simulink model "phantomx_sim_attitude"  (R2025b)
settings: Solver=daessc  StartTime=0.0  StopTime=20  RelTol=1e-3
InitFcn:
  | % Parametri del filtro
  | num_filters = 18;       % Numero di filtri in parallelo (i tuoi 18 giunti/segnali)
  | if evalin('base','exist(''tau_filtro'',''var'')')
  |     tau = evalin('base','tau_filtro');
  | else
  |     tau = 0.05; % costante di tempo del polo
  | end
  | a = 1 / tau;            % Polo del sistema
  | 
  | % 1. Creazione delle Matrici di Stato (State-Space)
  | % Matrice A (Dinamica del sistema): Diagonale con i poli
  | A = -a * eye(num_filters);
  | 
  | % Matrice B (Matrice di ingresso): Diagonale per mappare ogni input al suo stato
  | B = a * eye(num_filters);
  | 
  | % Matrice C (Matrice di uscita): Identità (vogliamo leggere gli stati direttamente)
  | C = eye(num_filters);
  | 
  | % Matrice D (Feedforward): Matrice di zeri (nessun collegamento diretto input-output)
  | D = zeros(num_filters, num_filters);
  | 
  | % 2. Creazione dell'oggetto State-Space in MATLAB
  | sys_filter = ss(A, B, C, D);
  | 
  | % Aggiungiamo i nomi per tenere tutto in ordine (opzionale ma consigliato)
  | sys_filter.InputName = strcat('Action_In_', string(1:num_filters));
  | sys_filter.OutputName = strcat('Filtered_Action_Out_', string(1:num_filters));
  | sys_filter.StateName = strcat('State_', string(1:num_filters));
  | 
  | % Mostra le proprietà del sistema creato
  | disp('Sistema State-Space creato con successo:');
  | sys_filter
  | 
  | run init_gait.m
values from neighbouring files (symbols this model uses):
  c2_par = [double(cfg.c2.attiva),            cfg.c2.z_nom,            cfg.c2.v_search,            cfg.c2.z_ext_max,            cfg.c2.t_reset,            cfg.c2.tol]    [init_gait.m]
  c2_soglia = inf    [init_gait.m]
undefined symbols (not defined in the file or in its folder): gait, X, Y, Z
libraries: sm_lib x305, nesl_utility x100, robotmaniplib x1, slpidlib x1
(part 1 of 5)
settings Model: Creator=andri  LastModifiedBy=eros2
settings SimscapeCC: SimscapeLogType=all  SimscapeLogLimitData=off

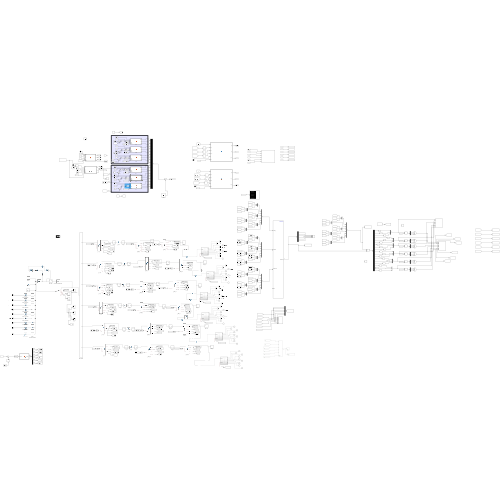
[thumbnail: Simulink's stored preview of the top-level diagram]
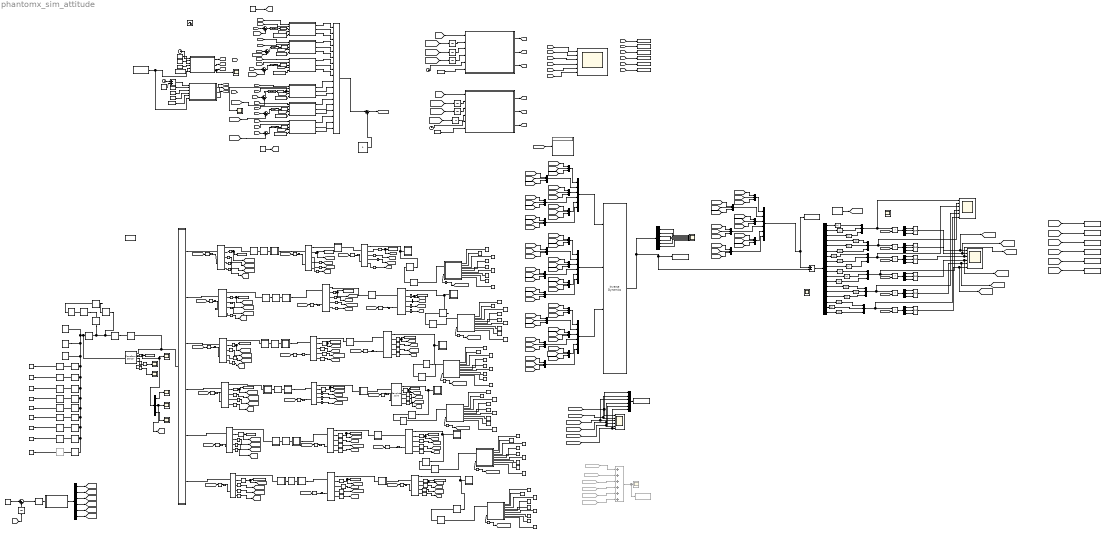
== system phantomx_sim_attitude ==
  note: LEFT
  note: RIGHT
  6-DOF Joint : sm_lib/Joints/6-DOF Joint  JointMode=Normal  CompositeWrenchDir=FollowerOnBase  CompositeWrenchFrame=BaseFrame  SenseConstraintForce=off  SenseConstraintTorque=off  SenseTotalForce=off  SenseTotalTorque=off  PxPositionTargetSpecify=off  PxPositionTargetPriority=High  PxPositionTargetValue=0  PxPositionTargetValueUnits=m  PxVelocityTargetSpecify=off  PxVelocityTargetPriority=High  PxVelocityTargetValue=0  PxVelocityTargetValueUnits=m/s  PxEquilibriumPosition=0  PxEquilibriumPositionUnits=m  PxSpringStiffness=0  PxSpringStiffnessUnits=N/m  PxDampingCoefficient=0  PxDampingCoefficientUnits=N/(m/s)  PxLowerLimitSpecify=off  PxLowerLimitBound=-1  PxLowerLimitBoundUnits=m  PxLowerLimitStiffness=1e6  PxLowerLimitStiffnessUnits=N/m  PxLowerLimitDamping=1e3  PxLowerLimitDampingUnits=N/(m/s)  PxLowerLimitTransitionRegionWidth=1e-4  PxLowerLimitTransitionRegionWidthUnits=m  PxUpperLimitSpecify=off  PxUpperLimitBound=1  PxUpperLimitBoundUnits=m  PxUpperLimitStiffness=1e6  PxUpperLimitStiffnessUnits=N/m  PxUpperLimitDamping=1e3  PxUpperLimitDampingUnits=N/(m/s)  PxUpperLimitTransitionRegionWidth=1e-4  PxUpperLimitTransitionRegionWidthUnits=m  PxTorqueActuationMode=NoTorque  PxMotionActuationMode=ComputedMotion  PxSensePosition=off  PxSenseVelocity=off  PxSenseAcceleration=off  PxSenseTorqueForce=off  PxSenseLowerLimitTorqueForce=off  PxSenseUpperLimitTorqueForce=off  PyPositionTargetSpecify=off  PyPositionTargetPriority=High  PyPositionTargetValue=0  PyPositionTargetValueUnits=m  PyVelocityTargetSpecify=off  PyVelocityTargetPriority=High  PyVelocityTargetValue=0  PyVelocityTargetValueUnits=m/s  PyEquilibriumPosition=0  PyEquilibriumPositionUnits=m  PySpringStiffness=0  PySpringStiffnessUnits=N/m  PyDampingCoefficient=0  PyDampingCoefficientUnits=N/(m/s)  PyLowerLimitSpecify=off  PyLowerLimitBound=-1  PyLowerLimitBoundUnits=m  PyLowerLimitStiffness=1e6  PyLowerLimitStiffnessUnits=N/m  PyLowerLimitDamping=1e3  PyLowerLimitDampingUnits=N/(m/s)  PyLowerLimitTransitionRegionWidth=1e-4  PyLowerLimitTransitionRegionWidthUnits=m  PyUpperLimitSpecify=off  PyUpperLimitBound=1  PyUpperLimitBoundUnits=m  PyUpperLimitStiffness=1e6  PyUpperLimitStiffnessUnits=N/m  PyUpperLimitDamping=1e3  PyUpperLimitDampingUnits=N/(m/s)  PyUpperLimitTransitionRegionWidth=1e-4  PyUpperLimitTransitionRegionWidthUnits=m  PyTorqueActuationMode=NoTorque  PyMotionActuationMode=ComputedMotion  PySensePosition=off  PySenseVelocity=off  PySenseAcceleration=off  PySenseTorqueForce=off  PySenseLowerLimitTorqueForce=off  PySenseUpperLimitTorqueForce=off  PzPositionTargetSpecify=on  PzPositionTargetPriority=High  PzPositionTargetValue=body_z0  PzPositionTargetValueUnits=m  PzVelocityTargetSpecify=off  PzVelocityTargetPriority=High  PzVelocityTargetValue=0  PzVelocityTargetValueUnits=m/s  PzEquilibriumPosition=0  PzEquilibriumPositionUnits=m  PzSpringStiffness=0  PzSpringStiffnessUnits=N/m  PzDampingCoefficient=0  PzDampingCoefficientUnits=N/(m/s)  PzLowerLimitSpecify=off  PzLowerLimitBound=-1  PzLowerLimitBoundUnits=m  PzLowerLimitStiffness=1e6  PzLowerLimitStiffnessUnits=N/m  PzLowerLimitDamping=1e3  PzLowerLimitDampingUnits=N/(m/s)  PzLowerLimitTransitionRegionWidth=1e-4  PzLowerLimitTransitionRegionWidthUnits=m  PzUpperLimitSpecify=off  PzUpperLimitBound=1  PzUpperLimitBoundUnits=m  PzUpperLimitStiffness=1e6  PzUpperLimitStiffnessUnits=N/m  PzUpperLimitDamping=1e3  PzUpperLimitDampingUnits=N/(m/s)  PzUpperLimitTransitionRegionWidth=1e-4  PzUpperLimitTransitionRegionWidthUnits=m  PzTorqueActuationMode=NoTorque  PzMotionActuationMode=ComputedMotion  PzSensePosition=off  PzSenseVelocity=off  PzSenseAcceleration=off  PzSenseTorqueForce=off  PzSenseLowerLimitTorqueForce=off  PzSenseUpperLimitTorqueForce=off  SphPositionTargetSpecify=off  SphPositionTargetPriority=High  SphPositionTargetRotationMethod=None  SphPositionTargetFollAlignAxisA=+X  SphPositionTargetBaseAlignAxisA=+Y  SphPositionTargetFollAlignAxisB=+Y  SphPositionTargetBaseAlignAxisB=+Z  SphPositionTargetRotationStandardAxis=+Z  SphPositionTargetRotationAngle=0  SphPositionTargetRotationAngleUnits=deg  SphPositionTargetRotationArbitraryAxis=[0 0 1]  SphPositionTargetRotationSequenceAxes=FollowerAxes  SphPositionTargetRotationSequence=XYX  SphPositionTargetRotationSequenceAngles=[0 0 0]  SphPositionTargetRotationSequenceAnglesUnits=deg  SphPositionTargetRotationMatrix=[1 0 0;0 1 0;0 0 1]  SphPositionTargetQuaternion=[1 0 0 0]  SphVelocityTargetSpecify=off  SphVelocityTargetPriority=High  SphVelocityTargetValue=[0 0 0]  SphVelocityTargetValueUnits=deg/s  SphVelocityTargetInFollowerFrame=on  SphEqPosRotationMethod=None  SphEqPosFollAlignAxisA=+X  SphEqPosBaseAlignAxisA=+Y  SphEqPosFollAlignAxisB=+Y  SphEqPosBaseAlignAxisB=+Z  SphEqPosRotationStandardAxis=+Z  SphEqPosRotationAngle=0  SphEqPosRotationAngleUnits=deg  SphEqPosRotationArbitraryAxis=[0 0 1]  SphEqPosRotationSequenceAxes=FollowerAxes  SphEqPosRotationSequence=XYX  SphEqPosRotationSequenceAngles=[0 0 0]  SphEqPosRotationSequenceAnglesUnits=deg  SphEqPosRotationMatrix=[1 0 0;0 1 0;0 0 1]  SphEqPosQuaternion=[1 0 0 0]  SphSpringStiffness=0  SphSpringStiffnessUnits=N*m/deg  SphDampingCoefficient=0  SphDampingCoefficientUnits=N*m/(deg/s)  SphLowerLimitSpecify=off  SphLowerLimitBound=15  SphLowerLimitBoundUnits=deg  SphLowerLimitStiffness=1e4  SphLowerLimitStiffnessUnits=N*m/deg  SphLowerLimitDamping=10  SphLowerLimitDampingUnits=N*m/(deg/s)  SphLowerLimitTransitionRegionWidth=0.1  SphLowerLimitTransitionRegionWidthUnits=deg  SphUpperLimitSpecify=off  SphUpperLimitBound=45  SphUpperLimitBoundUnits=deg  SphUpperLimitStiffness=1e4  SphUpperLimitStiffnessUnits=N*m/deg  SphUpperLimitDamping=10  SphUpperLimitDampingUnits=N*m/(deg/s)  SphUpperLimitTransitionRegionWidth=0.1  SphUpperLimitTransitionRegionWidthUnits=deg  SphTorqueActuationMode=NoTorque  SphActuateTorqueX=off  SphActuateTorqueY=off  SphActuateTorqueZ=off  SphActuateTorque=off  SphActuationFrame=BaseFrame  SphSensePosition=off  SphSenseVelocityX=off  SphSenseVelocityY=off  SphSenseVelocityZ=off  SphSenseVelocity=off  SphSenseAccelerationX=off  SphSenseAccelerationY=off  SphSenseAccelerationZ=off  SphSenseAcceleration=off  SphSenseLowerLimitTorqueMag=off  SphSenseUpperLimitTorqueMag=off  SphSensingFrame=BaseFrame
  6-DOF Joint1 : sm_lib/Joints/6-DOF Joint  JointMode=Normal  CompositeWrenchDir=FollowerOnBase  CompositeWrenchFrame=BaseFrame  SenseConstraintForce=off  SenseConstraintTorque=off  SenseTotalForce=off  SenseTotalTorque=off  PxPositionTargetSpecify=off  PxPositionTargetPriority=High  PxPositionTargetValue=0  PxPositionTargetValueUnits=m  PxVelocityTargetSpecify=off  PxVelocityTargetPriority=High  PxVelocityTargetValue=0  PxVelocityTargetValueUnits=m/s  PxEquilibriumPosition=0  PxEquilibriumPositionUnits=m  PxSpringStiffness=0  PxSpringStiffnessUnits=N/m  PxDampingCoefficient=0  PxDampingCoefficientUnits=N/(m/s)  PxLowerLimitSpecify=off  PxLowerLimitBound=-1  PxLowerLimitBoundUnits=m  PxLowerLimitStiffness=1e6  PxLowerLimitStiffnessUnits=N/m  PxLowerLimitDamping=1e3  PxLowerLimitDampingUnits=N/(m/s)  PxLowerLimitTransitionRegionWidth=1e-4  PxLowerLimitTransitionRegionWidthUnits=m  PxUpperLimitSpecify=off  PxUpperLimitBound=1  PxUpperLimitBoundUnits=m  PxUpperLimitStiffness=1e6  PxUpperLimitStiffnessUnits=N/m  PxUpperLimitDamping=1e3  PxUpperLimitDampingUnits=N/(m/s)  PxUpperLimitTransitionRegionWidth=1e-4  PxUpperLimitTransitionRegionWidthUnits=m  PxTorqueActuationMode=NoTorque  PxMotionActuationMode=ComputedMotion  PxSensePosition=off  PxSenseVelocity=off  PxSenseAcceleration=off  PxSenseTorqueForce=off  PxSenseLowerLimitTorqueForce=off  PxSenseUpperLimitTorqueForce=off  PyPositionTargetSpecify=off  PyPositionTargetPriority=High  PyPositionTargetValue=0  PyPositionTargetValueUnits=m  PyVelocityTargetSpecify=off  PyVelocityTargetPriority=High  PyVelocityTargetValue=0  PyVelocityTargetValueUnits=m/s  PyEquilibriumPosition=0  PyEquilibriumPositionUnits=m  PySpringStiffness=0  PySpringStiffnessUnits=N/m  PyDampingCoefficient=0  PyDampingCoefficientUnits=N/(m/s)  PyLowerLimitSpecify=off  PyLowerLimitBound=-1  PyLowerLimitBoundUnits=m  PyLowerLimitStiffness=1e6  PyLowerLimitStiffnessUnits=N/m  PyLowerLimitDamping=1e3  PyLowerLimitDampingUnits=N/(m/s)  PyLowerLimitTransitionRegionWidth=1e-4  PyLowerLimitTransitionRegionWidthUnits=m  PyUpperLimitSpecify=off  PyUpperLimitBound=1  PyUpperLimitBoundUnits=m  PyUpperLimitStiffness=1e6  PyUpperLimitStiffnessUnits=N/m  PyUpperLimitDamping=1e3  PyUpperLimitDampingUnits=N/(m/s)  PyUpperLimitTransitionRegionWidth=1e-4  PyUpperLimitTransitionRegionWidthUnits=m  PyTorqueActuationMode=NoTorque  PyMotionActuationMode=ComputedMotion  PySensePosition=off  PySenseVelocity=off  PySenseAcceleration=off  PySenseTorqueForce=off  PySenseLowerLimitTorqueForce=off  PySenseUpperLimitTorqueForce=off  PzPositionTargetSpecify=on  PzPositionTargetPriority=High  PzPositionTargetValue=body_z0  PzPositionTargetValueUnits=m  PzVelocityTargetSpecify=off  PzVelocityTargetPriority=High  PzVelocityTargetValue=0  PzVelocityTargetValueUnits=m/s  PzEquilibriumPosition=0  PzEquilibriumPositionUnits=m  PzSpringStiffness=0  PzSpringStiffnessUnits=N/m  PzDampingCoefficient=0  PzDampingCoefficientUnits=N/(m/s)  PzLowerLimitSpecify=off  PzLowerLimitBound=-1  PzLowerLimitBoundUnits=m  PzLowerLimitStiffness=1e6  PzLowerLimitStiffnessUnits=N/m  PzLowerLimitDamping=1e3  PzLowerLimitDampingUnits=N/(m/s)  PzLowerLimitTransitionRegionWidth=1e-4  PzLowerLimitTransitionRegionWidthUnits=m  PzUpperLimitSpecify=off  PzUpperLimitBound=1  PzUpperLimitBoundUnits=m  PzUpperLimitStiffness=1e6  PzUpperLimitStiffnessUnits=N/m  PzUpperLimitDamping=1e3  PzUpperLimitDampingUnits=N/(m/s)  PzUpperLimitTransitionRegionWidth=1e-4  PzUpperLimitTransitionRegionWidthUnits=m  PzTorqueActuationMode=NoTorque  PzMotionActuationMode=ComputedMotion  PzSensePosition=off  PzSenseVelocity=off  PzSenseAcceleration=off  PzSenseTorqueForce=off  PzSenseLowerLimitTorqueForce=off  PzSenseUpperLimitTorqueForce=off  SphPositionTargetSpecify=off  SphPositionTargetPriority=High  SphPositionTargetRotationMethod=None  SphPositionTargetFollAlignAxisA=+X  SphPositionTargetBaseAlignAxisA=+Y  SphPositionTargetFollAlignAxisB=+Y  SphPositionTargetBaseAlignAxisB=+Z  SphPositionTargetRotationStandardAxis=+Z  SphPositionTargetRotationAngle=0  SphPositionTargetRotationAngleUnits=deg  SphPositionTargetRotationArbitraryAxis=[0 0 1]  SphPositionTargetRotationSequenceAxes=FollowerAxes  SphPositionTargetRotationSequence=XYX  SphPositionTargetRotationSequenceAngles=[0 0 0]  SphPositionTargetRotationSequenceAnglesUnits=deg  SphPositionTargetRotationMatrix=[1 0 0;0 1 0;0 0 1]  SphPositionTargetQuaternion=[1 0 0 0]  SphVelocityTargetSpecify=off  SphVelocityTargetPriority=High  SphVelocityTargetValue=[0 0 0]  SphVelocityTargetValueUnits=deg/s  SphVelocityTargetInFollowerFrame=on  SphEqPosRotationMethod=None  SphEqPosFollAlignAxisA=+X  SphEqPosBaseAlignAxisA=+Y  SphEqPosFollAlignAxisB=+Y  SphEqPosBaseAlignAxisB=+Z  SphEqPosRotationStandardAxis=+Z  SphEqPosRotationAngle=0  SphEqPosRotationAngleUnits=deg  SphEqPosRotationArbitraryAxis=[0 0 1]  SphEqPosRotationSequenceAxes=FollowerAxes  SphEqPosRotationSequence=XYX  SphEqPosRotationSequenceAngles=[0 0 0]  SphEqPosRotationSequenceAnglesUnits=deg  SphEqPosRotationMatrix=[1 0 0;0 1 0;0 0 1]  SphEqPosQuaternion=[1 0 0 0]  SphSpringStiffness=0  SphSpringStiffnessUnits=N*m/deg  SphDampingCoefficient=0  SphDampingCoefficientUnits=N*m/(deg/s)  SphLowerLimitSpecify=off  SphLowerLimitBound=15  SphLowerLimitBoundUnits=deg  SphLowerLimitStiffness=1e4  SphLowerLimitStiffnessUnits=N*m/deg  SphLowerLimitDamping=10  SphLowerLimitDampingUnits=N*m/(deg/s)  SphLowerLimitTransitionRegionWidth=0.1  SphLowerLimitTransitionRegionWidthUnits=deg  SphUpperLimitSpecify=off  SphUpperLimitBound=45  SphUpperLimitBoundUnits=deg  SphUpperLimitStiffness=1e4  SphUpperLimitStiffnessUnits=N*m/deg  SphUpperLimitDamping=10  SphUpperLimitDampingUnits=N*m/(deg/s)  SphUpperLimitTransitionRegionWidth=0.1  SphUpperLimitTransitionRegionWidthUnits=deg  SphTorqueActuationMode=NoTorque  SphActuateTorqueX=off  SphActuateTorqueY=off  SphActuateTorqueZ=off  SphActuateTorque=off  SphActuationFrame=BaseFrame  SphSensePosition=off  SphSenseVelocityX=off  SphSenseVelocityY=off  SphSenseVelocityZ=off  SphSenseVelocity=off  SphSenseAccelerationX=off  SphSenseAccelerationY=off  SphSenseAccelerationZ=off  SphSenseAcceleration=off  SphSenseLowerLimitTorqueMag=off  SphSenseUpperLimitTorqueMag=off  SphSensingFrame=BaseFrame
  Abs{,1..17} (18 alike) : Abs  SaturateOnIntegerOverflow=off
  Add : Sum
  Add1 : Sum  Commented=on  Inputs=++++++
  Brick Solid : sm_lib/Body Elements/Brick Solid  BrickDimensions=[0.2 0.2 0.2]  BrickDimensionsUnits=m  ExportEntireGeometry=on  InertiaType=CalculateFromGeometry  BasedOnType=Mass  Density=1000  DensityUnits=kg/m^3  Mass=1  MassUnits=kg  CenterOfMass=[0 0 0]  CenterOfMassUnits=m  MomentsOfInertia=[1 1 1]  MomentsOfInertiaUnits=kg*m^2  ProductsOfInertia=[0 0 0]  ProductsOfInertiaUnits=kg*m^2  GraphicType=FromGeometry  MarkerShape=Sphere  MarkerSize=10  GraphicVisPropType=SimpleVisualProperties  GraphicDiffuseColor=[0.5 0.5 0.5]  GraphicOpacity=1  GraphicSpecularColor=[0.5 0.5 0.5 1.0]  GraphicAmbientColor=[0.15 0.15 0.15 1.0]  GraphicEmissiveColor=[0.0 0.0 0.0 1.0]  GraphicShininess=75  DoExposeReferenceFrame=on  SerializedFrames=<Frames/>
  Brick Solid1 : sm_lib/Body Elements/Brick Solid  BrickDimensions=[0.3 0.3 0.1]  BrickDimensionsUnits=m  ExportEntireGeometry=on  InertiaType=CalculateFromGeometry  BasedOnType=Mass  Density=1000  DensityUnits=kg/m^3  Mass=0.1  MassUnits=kg  CenterOfMass=[0 0 0]  CenterOfMassUnits=m  MomentsOfInertia=[1 1 1]  MomentsOfInertiaUnits=kg*m^2  ProductsOfInertia=[0 0 0]  ProductsOfInertiaUnits=kg*m^2  GraphicType=FromGeometry  MarkerShape=Sphere  MarkerSize=10  GraphicVisPropType=SimpleVisualProperties  GraphicDiffuseColor=[0.5 0.5 0.5]  GraphicOpacity=1  GraphicSpecularColor=[0.5 0.5 0.5 1.0]  GraphicAmbientColor=[0.15 0.15 0.15 1.0]  GraphicEmissiveColor=[0.0 0.0 0.0 1.0]  GraphicShininess=75  DoExposeReferenceFrame=on  SerializedFrames=<Frames/>
  Clock{,1..3} (4 alike) : Clock
  Connection Label{,1,4..5,27,45,54} (7 alike) : ConnectionLabel  Label=pavimento
  Connection Label{10,23..25,34,49,58} (7 alike) : ConnectionLabel  Label=ostacolo3
  Connection Label{3,7,11,26,35,50,59} (7 alike) : ConnectionLabel  Label=rampa
  Connection Label{6,12..14,28,46,55} (7 alike) : ConnectionLabel  Label=ostacolo7
  Connection Label{8,15,17..18,29,47,56} (7 alike) : ConnectionLabel  Label=ostacolo2
  Connection Label{2,9,16,19,30,48,57} (7 alike) : ConnectionLabel  Label=ostacolo1
  Connection Label{20,31..33,36,51,60} (7 alike) : ConnectionLabel  Label=ostacolo4
  Connection Label{21,37..38,40,42,52,61} (7 alike) : ConnectionLabel  Label=ostacolo5
  Connection Label{22,39,41,43..44,53,62} (7 alike) : ConnectionLabel  Label=ostacolo6
  Constant : Constant  Value=c2_soglia
  Constant1 : Constant  Value=gait.duty
  Constant10 : Constant  Value=c2_par
  Constant11 : Constant  Value=c2_par
  Constant12 : Constant  Value=0
  Constant19 : Constant  Value=deg2rad(-135)
  Constant2 : Constant  Value=gait.T
  Constant20 : Constant  Value=deg2rad(-90)
  Constant21 : Constant  Value=deg2rad(-45)
  Constant22 : Constant  Value=-1
  Constant23 : Constant
  Constant25 : Constant  Value=deg2rad(135)
  Constant26 : Constant  Value=deg2rad(90)
  Constant27 : Constant  Value=deg2rad(45)
  Constant28 : Constant  Value=0.5
  Constant3 : Constant  Value=gait.S
  Constant4 : Constant  Value=gait.H
  Constant5 : Constant  Value=gait.z0
  Constant6 : Constant  Value=gait.T
  Constant7 : Constant  Value=gait.S
  Constant8 : Constant  Value=gait.H
  Constant9 : Constant  Value=gait.z0
  Data Store Memory : DataStoreMemory  Priority=1  DataStoreName=joint_vector  WriteAfterWriteMsg=warning  InitialValue=zeros(21,1)  ShowAdditionalParam=off  OutDataTypeStr=double
  Data Store Write : DataStoreWrite  Priority=2  DataStoreName=joint_vector  DataStoreElements=joint_vector  EnableIndexing=on  IndexOptions=Index vector (dialog)  Indices=1  OutputSizes=1
  Data Store Write1 : DataStoreWrite  Priority=2  DataStoreName=joint_vector  DataStoreElements=joint_vector  EnableIndexing=on  IndexOptions=Index vector (dialog)  Indices=2  OutputSizes=1
  Data Store Write10 : DataStoreWrite  Priority=2  DataStoreName=joint_vector  DataStoreElements=joint_vector  EnableIndexing=on  IndexOptions=Index vector (dialog)  Indices=11  OutputSizes=1
  Data Store Write11 : DataStoreWrite  Priority=2  DataStoreName=joint_vector  DataStoreElements=joint_vector  EnableIndexing=on  IndexOptions=Index vector (dialog)  Indices=12  OutputSizes=1
  Data Store Write12 : DataStoreWrite  Priority=2  DataStoreName=joint_vector  DataStoreElements=joint_vector  EnableIndexing=on  IndexOptions=Index vector (dialog)  Indices=13  OutputSizes=1
  Data Store Write13 : DataStoreWrite  Priority=2  DataStoreName=joint_vector  DataStoreElements=joint_vector  EnableIndexing=on  IndexOptions=Index vector (dialog)  Indices=14  OutputSizes=1
  Data Store Write14 : DataStoreWrite  Priority=2  DataStoreName=joint_vector  DataStoreElements=joint_vector  EnableIndexing=on  IndexOptions=Index vector (dialog)  Indices=15  OutputSizes=1
  Data Store Write15 : DataStoreWrite  Priority=2  DataStoreName=joint_vector  DataStoreElements=joint_vector  EnableIndexing=on  IndexOptions=Index vector (dialog)  Indices=16  OutputSizes=1
  Data Store Write16 : DataStoreWrite  Priority=2  DataStoreName=joint_vector  DataStoreElements=joint_vector  EnableIndexing=on  IndexOptions=Index vector (dialog)  Indices=17  OutputSizes=1
  Data Store Write17 : DataStoreWrite  Priority=2  DataStoreName=joint_vector  DataStoreElements=joint_vector  EnableIndexing=on  IndexOptions=Index vector (dialog)  Indices=18  OutputSizes=1
  Data Store Write18 : DataStoreWrite  Priority=2  DataStoreName=joint_vector  DataStoreElements=joint_vector  EnableIndexing=on  IndexOptions=Index vector (dialog)  Indices=[19,20,21]  OutputSizes=1
  Data Store Write2 : DataStoreWrite  Priority=2  DataStoreName=joint_vector  DataStoreElements=joint_vector  EnableIndexing=on  IndexOptions=Index vector (dialog)  Indices=3  OutputSizes=1
  Data Store Write3 : DataStoreWrite  Priority=2  DataStoreName=joint_vector  DataStoreElements=joint_vector  EnableIndexing=on  IndexOptions=Index vector (dialog)  Indices=4  OutputSizes=1
  Data Store Write4 : DataStoreWrite  Priority=2  DataStoreName=joint_vector  DataStoreElements=joint_vector  EnableIndexing=on  IndexOptions=Index vector (dialog)  Indices=5  OutputSizes=1
  Data Store Write5 : DataStoreWrite  Priority=2  DataStoreName=joint_vector  DataStoreElements=joint_vector  EnableIndexing=on  IndexOptions=Index vector (dialog)  Indices=6  OutputSizes=1
  Data Store Write6 : DataStoreWrite  Priority=2  DataStoreName=joint_vector  DataStoreElements=joint_vector  EnableIndexing=on  IndexOptions=Index vector (dialog)  Indices=7  OutputSizes=1
  Data Store Write7 : DataStoreWrite  Priority=2  DataStoreName=joint_vector  DataStoreElements=joint_vector  EnableIndexing=on  IndexOptions=Index vector (dialog)  Indices=8  OutputSizes=1
  Data Store Write8 : DataStoreWrite  Priority=2  DataStoreName=joint_vector  DataStoreElements=joint_vector  EnableIndexing=on  IndexOptions=Index vector (dialog)  Indices=9  OutputSizes=1
  Data Store Write9 : DataStoreWrite  Priority=2  DataStoreName=joint_vector  DataStoreElements=joint_vector  EnableIndexing=on  IndexOptions=Index vector (dialog)  Indices=10  OutputSizes=1
  Demux : Demux  Outputs=[3,3,3,3,3,3]
  Demux1 : Demux  Outputs=18
  Demux{2..8} (7 alike) : Demux  Outputs=3
  Demux9 : Demux  Outputs=6
  Display : Display
  FL : MATLAB Function  TreatAsAtomicUnit=on
  FR : MATLAB Function  TreatAsAtomicUnit=on
  From127 : From  Commented=on  GotoTag=Force_sens_lf
  From128 : From  Commented=on  GotoTag=Force_sens_lm
  From129 : From  Commented=on  GotoTag=Force_sens_lr
  From130 : From  Commented=on  GotoTag=Force_sens_rf
  From131 : From  Commented=on  GotoTag=Force_sens_rm
  From132 : From  Commented=on  GotoTag=Force_sens_rr
  Inverse Dynamics : robotmaniplib/Inverse Dynamics  RigidBodyTree=robotModel  SimulateUsing=Interpreted execution
  MATLAB Function : MATLAB Function  TreatAsAtomicUnit=on
  MATLAB Function1 : MATLAB Function  TreatAsAtomicUnit=on
  MATLAB Function2 : MATLAB Function  TreatAsAtomicUnit=on
  MATLAB Function3 : MATLAB Function  TreatAsAtomicUnit=on
  MATLAB Function4 : MATLAB Function  TreatAsAtomicUnit=on
  ML : MATLAB Function  TreatAsAtomicUnit=on
  MP_BODY : Subsystem
  MR : MATLAB Function  TreatAsAtomicUnit=on
  MechanismConfiguration : sm_lib/Utilities/Mechanism Configuration  UniformGravity=Constant  GravityVector=[0 0 -9.81]  GravityVectorUnits=m/s^2  LinearizationDelta=0.001  JointModeTransitionNonlinearIterations=2
  Mux{,1..3} (4 alike) : Mux  Inputs=[3,3,3,3,3,3]
  Mux{4..7,9..34} (30 alike) : Mux  Inputs=3
  Mux35 : Mux  Inputs=6
  Mux8 : Mux  Inputs=18
  OR{,1..5} (6 alike) : Logic  Operator=OR  Inputs=3  IconShape=distinctive  AllPortsSameDT=off  OutDataTypeStr=boolean
  PID Controller : slpidlib/PID Controller  Controller=PID  Form=Parallel  TimeDomain=Discrete-time  UseExternalTs=off  SampleTime=0.001  IntegratorMethod=Forward Euler  FilterMethod=Forward Euler  ControllerParametersSource=internal  P=30  I=0  UseKiTs=off  D=0  UseExternalDerivativeSource=off  N=100  UseFilter=on  TunerSelectOption=Transfer Function Based (PID Tuner App)  InitialConditionSource=internal  InitialConditionForIntegrator=0  InitialConditionForFilter=0  DifferentiatorICPrevScaledInput=0  ExternalReset=none  TrackingMode=off  Kt=1  LimitOutput=off  SatLimitsSource=internal  UpperSaturationLimit=inf  LowerSaturationLimit=-inf  LinearizeAsGain=on  AntiWindupMode=none  Kb=1  LimitIntegrator=off  UpperIntegratorSaturationLimit=inf  LowerIntegratorSaturationLimit=-inf  POutMin=[]  POutMax=[]  IOutMin=[]  IOutMax=[]  DOutMin=[]  DOutMax=[]  NOutMin=[]  NOutMax=[]  SumOutMin=[]  SumOutMax=[]  SaturationOutMin=[]  SaturationOutMax=[]  PParamMin=[]  PParamMax=[]  IParamMin=[]  IParamMax=[]  DParamMin=[]  DParamMax=[]  NParamMin=[]  NParamMax=[]  KbParamMin=[]  KbParamMax=[]  KtParamMin=[]  KtParamMax=[]  KbOutMin=[]  KbOutMax=[]  KtOutMin=[]  KtOutMax=[]  IntegratorOutMin=[]  IntegratorOutMax=[]  FilterOutMin=[]  FilterOutMax=[]  SumI1OutMin=[]  SumI1OutMax=[]  SumI2OutMin=[]  SumI2OutMax=[]  SumI3OutMin=[]  SumI3OutMax=[]  SumI4OutMin=[]  SumI4OutMax=[]  SumDOutMin=[]  SumDOutMax=[]  DifferentiatorOutMin=[]  DifferentiatorOutMax=[]  FilterDiffOutCoefMin=[]  FilterDiffOutCoefMax=[]  ReciprocalOutMin=[]  ReciprocalOutMax=[]  SumDenOutMin=[]  SumDenOutMax=[]  SumNumOutMin=[]  SumNumOutMax=[]  DivideOutMin=[]  DivideOutMax=[]  UdiffTsProdOutMin=[]  UdiffTsProdOutMax=[]  NTsProdOutMin=[]  NTsProdOutMax=[]  UintegralTsProdOutMin=[]  UintegralTsProdOutMax=[]  UngainTsProdOutMin=[]  UngainTsProdOutMax=[]  ClampingZeroOutDataTypeStr=Inherit: Inherit via back propagation  ClampingZeroOutMin=[]  ClampingZeroOutMax=[]  FilterDenConstantOutDataTypeStr=Inherit: Inherit via back propagation  FilterDenConstantOutMin=[]  FilterDenConstantOutMax=[]  PCopyOutDataTypeStr=Inherit: Inherit via back propagation  PCopyOutMin=[]  PCopyOutMax=[]  NCopyOutDataTypeStr=Inherit: Inherit via back propagation  NCopyOutMin=[]  NCopyOutMax=[]  IntegratorContinuousStateAttributes=''  IntegratorStateMustResolveToSignalObject=off  IntegratorRTWStateStorageClass=Auto  FilterContinuousStateAttributes=''  FilterStateMustResolveToSignalObject=off  FilterRTWStateStorageClass=Auto  ParallelPVariant=InternalParameters  IdealPVariant=Disabled  IVariant=InternalParameters  DVariant=InternalParameters  IntegratorVariant=Discrete  SatVariant=Disabled  AWVariant=Passthrough  PCopyVariant=Disabled  TRVariant=Disabled  FdbkBlocksVariant=Forward  IdealPFdbkVariant=Disabled  SatFdbkVariant=Disabled  DerivativeFilterVariant=ForwardEulerFilter  NVariant=InternalParameters  NCopyVariant=Disabled  FilterICVariant=InternalICsFilter  IntegratorICVariant=InternalICs  ExternalResetVariant=Disabled  TRSumVariant=Passthrough  SumFdbkVariant=Disabled  SumVariant=Sum_PID  TsampFilterVariant=InternalTs  TsampNgainVariant=Passthrough  TsampIntegralVariant=Disabled_SignalSpec  ExternalSaturationOutDataTypeStr=Inherit: Same as second input  DerivativeSourceVariant=ErrorSignal  PreIntVariant=InternalPreInt
  PS-Simulink Converter{,2..80} (80 alike) : nesl_utility/PS-Simulink Converter  PhysicalDomain=network_engine_domain  SubClassName=ps_output  LeftPortType=input  RightPortType=output  PseudoPeriodic=off  Frequencies=[]  VectorFormat=inherit  Unit=inherit  AffineConversion=off
  PS-Simulink Converter1 : nesl_utility/PS-Simulink Converter  PhysicalDomain=network_engine_domain  SubClassName=ps_output  LeftPortType=input  RightPortType=output  PseudoPeriodic=off  Frequencies=[]  VectorFormat=1-D array  Unit=inherit  AffineConversion=off
  RL : MATLAB Function  TreatAsAtomicUnit=on
  RR : MATLAB Function  TreatAsAtomicUnit=on
  Rate Limiter{,1..5} (6 alike) : RateLimiter  RisingSlewLimit=0.3  FallingSlewLimit=-0.3  SampleTimeMode=inherited  InitialCondition=0.14
  Relational Operator{,1..5} (6 alike) : RelationalOperator  Operator=>  OutDataTypeStr=boolean  RndMeth=Simplest  InputSameDT=off
  Rigid Transform : sm_lib/Frames and Transforms/Rigid Transform  RotationMethod=None  FollAlignAxisA=+X  BaseAlignAxisA=+Y  FollAlignAxisB=+Y  BaseAlignAxisB=+Z  RotationStandardAxis=+Y  RotationAngle=4  RotationAngleUnits=deg  RotationArbitraryAxis=[0 0 1]  RotationSequenceAxes=FollowerAxes  RotationSequence=XYX  RotationSequenceAngles=[0 0 0]  RotationSequenceAnglesUnits=deg  RotationMatrix=[1 0 0;0 1 0;0 0 1]  Quaternion=[1 0 0 0]  TranslationMethod=Cartesian  TranslationCartesianOffset=[0,0,0.05]  TranslationCartesianOffsetUnits=m  TranslationStandardAxis=+Z  TranslationStandardOffset=0  TranslationStandardOffsetUnits=m  TranslationROffset=0  TranslationROffsetUnits=m  TranslationThetaOffset=0  TranslationThetaOffsetUnits=deg  TranslationZOffset=0  TranslationZOffsetUnits=m
  Rigid Transform{1..6} (6 alike) : sm_lib/Frames and Transforms/Rigid Transform  RotationMethod=None  FollAlignAxisA=+X  BaseAlignAxisA=+Y  FollAlignAxisB=+Y  BaseAlignAxisB=+Z  RotationStandardAxis=+Z  RotationAngle=0  RotationAngleUnits=deg  RotationArbitraryAxis=[0 0 1]  RotationSequenceAxes=FollowerAxes  RotationSequence=XYX  RotationSequenceAngles=[0 0 0]  RotationSequenceAnglesUnits=deg  RotationMatrix=[1 0 0;0 1 0;0 0 1]  Quaternion=[1 0 0 0]  TranslationMethod=Cartesian  TranslationCartesianOffset=foot_xyz  TranslationCartesianOffsetUnits=m  TranslationStandardAxis=+Z  TranslationStandardOffset=0  TranslationStandardOffsetUnits=m  TranslationROffset=0  TranslationROffsetUnits=m  TranslationThetaOffset=0  TranslationThetaOffsetUnits=deg  TranslationZOffset=0  TranslationZOffsetUnits=m
  Rigid Transform{10..16} (7 alike) : sm_lib/Frames and Transforms/Rigid Transform  RotationMethod=None  FollAlignAxisA=+X  BaseAlignAxisA=+Y  FollAlignAxisB=+Y  BaseAlignAxisB=+Z  RotationStandardAxis=+Y  RotationAngle=4  RotationAngleUnits=deg  RotationArbitraryAxis=[0 0 1]  RotationSequenceAxes=FollowerAxes  RotationSequence=XYX  RotationSequenceAngles=[0 0 0]  RotationSequenceAnglesUnits=deg  RotationMatrix=[1 0 0;0 1 0;0 0 1]  Quaternion=[1 0 0 0]  TranslationMethod=Cartesian  TranslationCartesianOffset=floor_off  TranslationCartesianOffsetUnits=m  TranslationStandardAxis=+Z  TranslationStandardOffset=0  TranslationStandardOffsetUnits=m  TranslationROffset=0  TranslationROffsetUnits=m  TranslationThetaOffset=0  TranslationThetaOffsetUnits=deg  TranslationZOffset=0  TranslationZOffsetUnits=m
  Rigid Transform7 : sm_lib/Frames and Transforms/Rigid Transform  RotationMethod=None  FollAlignAxisA=+X  BaseAlignAxisA=+Y  FollAlignAxisB=+Y  BaseAlignAxisB=+Z  RotationStandardAxis=+Y  RotationAngle=4  RotationAngleUnits=deg  RotationArbitraryAxis=[0 0 1]  RotationSequenceAxes=FollowerAxes  RotationSequence=XYX  RotationSequenceAngles=[0 0 0]  RotationSequenceAnglesUnits=deg  RotationMatrix=[1 0 0;0 1 0;0 0 1]  Quaternion=[1 0 0 0]  TranslationMethod=Cartesian  TranslationCartesianOffset=[0,0,-0.4]  TranslationCartesianOffsetUnits=m  TranslationStandardAxis=+Z  TranslationStandardOffset=0  TranslationStandardOffsetUnits=m  TranslationROffset=0  TranslationROffsetUnits=m  TranslationThetaOffset=0  TranslationThetaOffsetUnits=deg  TranslationZOffset=0  TranslationZOffsetUnits=m
  Rigid Transform_Rampa : sm_lib/Frames and Transforms/Rigid Transform  RotationMethod=StandardAxis  FollAlignAxisA=+X  BaseAlignAxisA=+Y  FollAlignAxisB=+Y  BaseAlignAxisB=+Z  RotationStandardAxis=+Y  RotationAngle=8  RotationAngleUnits=deg  RotationArbitraryAxis=[0 0 1]  RotationSequenceAxes=FollowerAxes  RotationSequence=XYX  RotationSequenceAngles=[0 0 0]  RotationSequenceAnglesUnits=deg  RotationMatrix=[1 0 0;0 1 0;0 0 1]  Quaternion=[1 0 0 0]  TranslationMethod=Cartesian  TranslationCartesianOffset=[-1.15358 0 0.141854]  TranslationCartesianOffsetUnits=m  TranslationStandardAxis=+Z  TranslationStandardOffset=0  TranslationStandardOffsetUnits=m  TranslationROffset=0  TranslationROffsetUnits=m  TranslationThetaOffset=0  TranslationThetaOffsetUnits=deg  TranslationZOffset=0  TranslationZOffsetUnits=m
  Saturation{,1..5} (6 alike) : Saturate  LowerLimit=0.07
  Scope{,2..3,6,8} (5 alike) : Scope  NumInputPorts=6
      Scope settings: ActiveDisplayYMinimum=-0.97490857176413459  ActiveDisplayYMaximum=0.98281108617034962  DataLoggingVariableName=ScopeData3
      Scope2 settings: ActiveDisplayYMinimum=-0.12499999999999997  ActiveDisplayYMaximum=1.125  DataLoggingVariableName=ScopeData5
      Scope3 settings: ActiveDisplayYMinimum=-1.0416972330414633  ActiveDisplayYMaximum=9.3752750973731729  DataLoggingVariableName=ScopeData6
      Scope6 settings: ActiveDisplayYMinimum=-1.2196121679450986  ActiveDisplayYMaximum=10.97650975309802  DataLoggingVariableName=ScopeData9
      Scope8 settings: ActiveDisplayYMinimum=0.08108  ActiveDisplayYMaximum=0.17028000000000013  DataLoggingVariableName=ScopeData11
  Scope{1,5,7,9} (4 alike) : Scope
      Scope1 settings: ActiveDisplayYMinimum=-1  ActiveDisplayYMaximum=1  DataLoggingVariableName=ScopeData4
      Scope5 settings: DataLoggingVariableName=ScopeData8
      Scope7 settings: ActiveDisplayYMinimum=0.087712862318840581  ActiveDisplayYMaximum=0.14206068840579711  DataLoggingVariableName=ScopeData10
      Scope9 settings: ActiveDisplayYMinimum=0.10908427867678951  ActiveDisplayYMaximum=0.1791562743785256  DataLoggingVariableName=ScopeData15
  Scope4 : Scope  Commented=on
      settings: ActiveDisplayYMinimum=12.945948389596449  ActiveDisplayYMaximum=24.868135963555797  DataLoggingVariableName=ScopeData7
  Selector : Selector  InputPortWidth=18  IndexOptions=Index vector (dialog)  Indices=1  OutputSizes=1
  Selector1 : Selector  InputPortWidth=18  IndexOptions=Index vector (dialog)  Indices=2  OutputSizes=1
  Selector10 : Selector  InputPortWidth=18  IndexOptions=Index vector (dialog)  Indices=17  OutputSizes=1
  Selector11 : Selector  InputPortWidth=18  IndexOptions=Index vector (dialog)  Indices=14  OutputSizes=1
  Selector12 : Selector  InputPortWidth=18  IndexOptions=Index vector (dialog)  Indices=11  OutputSizes=1
  Selector13 : Selector  InputPortWidth=18  IndexOptions=Index vector (dialog)  Indices=8  OutputSizes=1
  Selector14 : Selector  InputPortWidth=18  IndexOptions=Index vector (dialog)  Indices=9  OutputSizes=1
  Selector15 : Selector  InputPortWidth=18  IndexOptions=Index vector (dialog)  Indices=12  OutputSizes=1
  Selector16 : Selector  InputPortWidth=18  IndexOptions=Index vector (dialog)  Indices=15  OutputSizes=1
  Selector17 : Selector  InputPortWidth=18  IndexOptions=Index vector (dialog)  Indices=18  OutputSizes=1
  Selector2 : Selector  InputPortWidth=18  IndexOptions=Index vector (dialog)  Indices=3  OutputSizes=1
  Selector3 : Selector  InputPortWidth=18  IndexOptions=Index vector (dialog)  Indices=4  OutputSizes=1
  Selector4 : Selector  InputPortWidth=18  IndexOptions=Index vector (dialog)  Indices=5  OutputSizes=1
  Selector5 : Selector  InputPortWidth=18  IndexOptions=Index vector (dialog)  Indices=6  OutputSizes=1
  Selector6 : Selector  InputPortWidth=18  IndexOptions=Index vector (dialog)  Indices=7  OutputSizes=1
  Selector7 : Selector  InputPortWidth=18  IndexOptions=Index vector (dialog)  Indices=10  OutputSizes=1
  Selector8 : Selector  InputPortWidth=18  IndexOptions=Index vector (dialog)  Indices=13  OutputSizes=1
  Selector9 : Selector  InputPortWidth=18  IndexOptions=Index vector (dialog)  Indices=16  OutputSizes=1
  Simulink-PS Converter{,1..9,18..25} (18 alike) : nesl_utility/Simulink-PS Converter  PhysicalDomain=network_engine_domain  SubClassName=ps_input  LeftPortType=input  RightPortType=output  PseudoPeriodic=off  Frequencies=[]  NoiseDistribution=none  NoiseParameters=[]  Unit=1  AffineConversion=off  FilteringAndDerivatives=filter  SimscapeFilterOrder=2  InputFilterTimeConstant=0.01  UdotUserProvided=0
  Sine Wave13 : Sin  Amplitude=0.07  SampleTime=0
  Solid_Ostacolo1 : sm_lib/Body Elements/File Solid  ExtGeomFileName=simscape\props\ProvaPianoImperfettoOstacolo.stl  UnitType=Custom  ExtGeomFileUnits=m  StepReaderType=HEX  ExportConvexHullGeometry=on  InertiaType=CalculateFromGeometry  BasedOnType=Mass  Density=1000  DensityUnits=kg/m^3  Mass=1  MassUnits=kg  CenterOfMass=[0 0 0]  CenterOfMassUnits=m  MomentsOfInertia=[1 1 1]  MomentsOfInertiaUnits=kg*m^2  ProductsOfInertia=[0 0 0]  ProductsOfInertiaUnits=kg*m^2  GraphicType=FromGeometry  MarkerShape=Sphere  MarkerSize=10  GraphicVisPropType=SimpleVisualProperties  GraphicDiffuseColor=[1 0.5 0.5]  GraphicOpacity=1  GraphicSpecularColor=[0.5 0.5 0.5 1.0]  GraphicAmbientColor=[0.15 0.15 0.15 1.0]  GraphicEmissiveColor=[0.0 0.0 0.0 1.0]  GraphicShininess=75  DoExposeReferenceFrame=on  SerializedFrames=<Frames/>
  Solid_Ostacolo2 : sm_lib/Body Elements/File Solid  ExtGeomFileName=simscape\props\ProvaPianoImperfettoOstacolo2.stl  UnitType=Custom  ExtGeomFileUnits=m  StepReaderType=HEX  ExportConvexHullGeometry=on  InertiaType=CalculateFromGeometry  BasedOnType=Mass  Density=1000  DensityUnits=kg/m^3  Mass=1  MassUnits=kg  CenterOfMass=[0 0 0]  CenterOfMassUnits=m  MomentsOfInertia=[1 1 1]  MomentsOfInertiaUnits=kg*m^2  ProductsOfInertia=[0 0 0]  ProductsOfInertiaUnits=kg*m^2  GraphicType=FromGeometry  MarkerShape=Sphere  MarkerSize=10  GraphicVisPropType=SimpleVisualProperties  GraphicDiffuseColor=[0.5 0.5 1]  GraphicOpacity=1  GraphicSpecularColor=[0.5 0.5 0.5 1.0]  GraphicAmbientColor=[0.15 0.15 0.15 1.0]  GraphicEmissiveColor=[0.0 0.0 0.0 1.0]  GraphicShininess=75  DoExposeReferenceFrame=on  SerializedFrames=<Frames/>
  Solid_Ostacolo3 : sm_lib/Body Elements/File Solid  ExtGeomFileName=simscape\props\ProvaPianoImperfettoOstacolo3.stl  UnitType=Custom  ExtGeomFileUnits=m  StepReaderType=HEX  ExportConvexHullGeometry=on  InertiaType=CalculateFromGeometry  BasedOnType=Mass  Density=1000  DensityUnits=kg/m^3  Mass=1  MassUnits=kg  CenterOfMass=[0 0 0]  CenterOfMassUnits=m  MomentsOfInertia=[1 1 1]  MomentsOfInertiaUnits=kg*m^2  ProductsOfInertia=[0 0 0]  ProductsOfInertiaUnits=kg*m^2  GraphicType=FromGeometry  MarkerShape=Sphere  MarkerSize=10  GraphicVisPropType=SimpleVisualProperties  GraphicDiffuseColor=[0.5 1 0.5]  GraphicOpacity=1  GraphicSpecularColor=[0.5 0.5 0.5 1.0]  GraphicAmbientColor=[0.15 0.15 0.15 1.0]  GraphicEmissiveColor=[0.0 0.0 0.0 1.0]  GraphicShininess=75  DoExposeReferenceFrame=on  SerializedFrames=<Frames/>
  Solid_Ostacolo4 : sm_lib/Body Elements/File Solid  ExtGeomFileName=simscape\props\ProvaPianoImperfettoOstacolo4.stl  UnitType=Custom  ExtGeomFileUnits=m  StepReaderType=HEX  ExportConvexHullGeometry=on  InertiaType=CalculateFromGeometry  BasedOnType=Mass  Density=1000  DensityUnits=kg/m^3  Mass=1  MassUnits=kg  CenterOfMass=[0 0 0]  CenterOfMassUnits=m  MomentsOfInertia=[1 1 1]  MomentsOfInertiaUnits=kg*m^2  ProductsOfInertia=[0 0 0]  ProductsOfInertiaUnits=kg*m^2  GraphicType=FromGeometry  MarkerShape=Sphere  MarkerSize=10  GraphicVisPropType=SimpleVisualProperties  GraphicDiffuseColor=[1 1 0.5]  GraphicOpacity=1  GraphicSpecularColor=[0.5 0.5 0.5 1.0]  GraphicAmbientColor=[0.15 0.15 0.15 1.0]  GraphicEmissiveColor=[0.0 0.0 0.0 1.0]  GraphicShininess=75  DoExposeReferenceFrame=on  SerializedFrames=<Frames/>
  Solid_Ostacolo5 : sm_lib/Body Elements/File Solid  ExtGeomFileName=simscape\props\ProvaPianoImperfettoOstacolo5.stl  UnitType=Custom  ExtGeomFileUnits=m  StepReaderType=HEX  ExportConvexHullGeometry=on  InertiaType=CalculateFromGeometry  BasedOnType=Mass  Density=1000  DensityUnits=kg/m^3  Mass=1  MassUnits=kg  CenterOfMass=[0 0 0]  CenterOfMassUnits=m  MomentsOfInertia=[1 1 1]  MomentsOfInertiaUnits=kg*m^2  ProductsOfInertia=[0 0 0]  ProductsOfInertiaUnits=kg*m^2  GraphicType=FromGeometry  MarkerShape=Sphere  MarkerSize=10  GraphicVisPropType=SimpleVisualProperties  GraphicDiffuseColor=[0.5 1 0.5]  GraphicOpacity=1  GraphicSpecularColor=[0.5 0.5 0.5 1.0]  GraphicAmbientColor=[0.15 0.15 0.15 1.0]  GraphicEmissiveColor=[0.0 0.0 0.0 1.0]  GraphicShininess=75  DoExposeReferenceFrame=on  SerializedFrames=<Frames/>
  Solid_Ostacolo6 : sm_lib/Body Elements/File Solid  ExtGeomFileName=simscape\props\ProvaPianoImperfettoOstacolo6.stl  UnitType=Custom  ExtGeomFileUnits=m  StepReaderType=HEX  ExportConvexHullGeometry=on  InertiaType=CalculateFromGeometry  BasedOnType=Mass  Density=1000  DensityUnits=kg/m^3  Mass=1  MassUnits=kg  CenterOfMass=[0 0 0]  CenterOfMassUnits=m  MomentsOfInertia=[1 1 1]  MomentsOfInertiaUnits=kg*m^2  ProductsOfInertia=[0 0 0]  ProductsOfInertiaUnits=kg*m^2  GraphicType=FromGeometry  MarkerShape=Sphere  MarkerSize=10  GraphicVisPropType=SimpleVisualProperties  GraphicDiffuseColor=[0.5 1 1]  GraphicOpacity=1  GraphicSpecularColor=[0.5 0.5 0.5 1.0]  GraphicAmbientColor=[0.15 0.15 0.15 1.0]  GraphicEmissiveColor=[0.0 0.0 0.0 1.0]  GraphicShininess=75  DoExposeReferenceFrame=on  SerializedFrames=<Frames/>
  Solid_Ostacolo7 : sm_lib/Body Elements/File Solid  ExtGeomFileName=simscape\props\ProvaPianoImperfettoOstacolo7.stl  UnitType=Custom  ExtGeomFileUnits=m  StepReaderType=HEX  ExportConvexHullGeometry=on  InertiaType=CalculateFromGeometry  BasedOnType=Mass  Density=1000  DensityUnits=kg/m^3  Mass=1  MassUnits=kg  CenterOfMass=[0 0 0]  CenterOfMassUnits=m  MomentsOfInertia=[1 1 1]  MomentsOfInertiaUnits=kg*m^2  ProductsOfInertia=[0 0 0]  ProductsOfInertiaUnits=kg*m^2  GraphicType=FromGeometry  MarkerShape=Sphere  MarkerSize=10  GraphicVisPropType=SimpleVisualProperties  GraphicDiffuseColor=[1 0.5 1]  GraphicOpacity=1  GraphicSpecularColor=[0.5 0.5 0.5 1.0]  GraphicAmbientColor=[0.15 0.15 0.15 1.0]  GraphicEmissiveColor=[0.0 0.0 0.0 1.0]  GraphicShininess=75  DoExposeReferenceFrame=on  SerializedFrames=<Frames/>
  Solid_Pavimento : sm_lib/Body Elements/File Solid  ExtGeomFileName=simscape\props\ProvaPianoImperfettoCube.stl  UnitType=Custom  ExtGeomFileUnits=m  StepReaderType=HEX  ExportConvexHullGeometry=on  InertiaType=CalculateFromGeometry  BasedOnType=Mass  Density=1000  DensityUnits=kg/m^3  Mass=1  MassUnits=kg  CenterOfMass=[0 0 0]  CenterOfMassUnits=m  MomentsOfInertia=[1 1 1]  MomentsOfInertiaUnits=kg*m^2  ProductsOfInertia=[0 0 0]  ProductsOfInertiaUnits=kg*m^2  GraphicType=FromGeometry  MarkerShape=Sphere  MarkerSize=10  GraphicVisPropType=SimpleVisualProperties  GraphicDiffuseColor=[0.5 0.5 0.5]  GraphicOpacity=1  GraphicSpecularColor=[0.5 0.5 0.5 1.0]  GraphicAmbientColor=[0.15 0.15 0.15 1.0]  GraphicEmissiveColor=[0.0 0.0 0.0 1.0]  GraphicShininess=75  DoExposeReferenceFrame=on  SerializedFrames=<Frames/>
  Solid_Rampa : sm_lib/Body Elements/File Solid  Commented=on  ExtGeomFileName=simscape\props\ProvaPianoImperfettoCube.stl  UnitType=Custom  ExtGeomFileUnits=m  StepReaderType=HEX  ExportConvexHullGeometry=on  InertiaType=CalculateFromGeometry  BasedOnType=Mass  Density=1000  DensityUnits=kg/m^3  Mass=1  MassUnits=kg  CenterOfMass=[0 0 0]  CenterOfMassUnits=m  MomentsOfInertia=[1 1 1]  MomentsOfInertiaUnits=kg*m^2  ProductsOfInertia=[0 0 0]  ProductsOfInertiaUnits=kg*m^2  GraphicType=FromGeometry  MarkerShape=Sphere  MarkerSize=10  GraphicVisPropType=SimpleVisualProperties  GraphicDiffuseColor=[0.5 0.5 0.5]  GraphicOpacity=1  GraphicSpecularColor=[0.5 0.5 0.5 1.0]  GraphicAmbientColor=[0.15 0.15 0.15 1.0]  GraphicEmissiveColor=[0.0 0.0 0.0 1.0]  GraphicShininess=75  DoExposeReferenceFrame=on  SerializedFrames=<Frames/>
  Solver Configuration : nesl_utility/Solver Configuration  PhysicalDomain=network_engine_domain  SubClassName=solver  LeftPortType=input  RightPortType=generic  Tones=[]  Harmonics=[]  SimulateNoise=off  Profile=off  UseLocalSampling=off  EnableSwitchedLinearOptims=on  FrequencyDomain=off  UseCCode=off  RelTol=0.001  AbsTol=0.001  MinStep=1e-09  ToWorkspace=off  RevertToSquareIcSolve=off  NumHomotopyIterations=100  PhasorMode=off  PhasorModeNumHarmonics=1  ConsistencySolver=NEWTON_XTOL_AFTER_FTOL  IndexReductionMethod=DerivativeReplacement  DoDC=off  ResidualTolerance=1e-09  ConsistencyTolSource=GLOBAL  ConsistencyAbsTol=0.001  ConsistencyRelTol=0.001  ConsistencyTolFactor=0.001  UseLocalSolver=off  LocalSolverChoice=NE_BACKWARD_EULER_ADVANCER  ResolveIndetEquations=on  FunctionEvalNumThread=1  LocalSolverSampleTime=0.001  DoFixedCost=off  MaxNonlinIter=3  MaxModeIter=2  ComputeImpulses=off  ImpulseIterations=2  LinearAlgebra=auto  LinearAlgebraNumThread=0  EquationFormulation=NE_TIME_EF  DelaysMemoryBudget=1024  AutomaticFiltering=on  FilteringTimeConstant=0.001  PartitionStorageMethod=AS_NEEDED  PartitionMemoryBudget=1024  PartitionMethod=ROBUST  MultibodyUseLocalSolver=on  MultibodyLocalSolverChoice=ODE1  MultibodyLocalSolverSampleTime=0.001
  Spatial Contact Force : sm_lib/Forces and Torques/Spatial Contact Force  SenseSeparationDistance=off  NormalForceType=SmoothSpringDamper  NormalStiffness=1200  NormalStiffnessUnits=N/m  NormalDamping=50  NormalDampingUnits=N/(m/s)  NormalTransitionRegionWidth=0.002  NormalTransitionRegionWidthUnits=m  FrictionType=SmoothStickSlip  CoefficientOfStaticFriction=0.5  CoefficientOfDynamicFriction=0.3  FrictionalCriticalVelocity=1e-3  FrictionalCriticalVelocityUnits=m/s  SenseContactSignal=off  SensePenetrationDepth=off  SenseNormalVelocity=off  SenseTangentialVelocity=off  SensingForceTorqueDirection=BaseOnFollower  SensingForceTorqueResolutionFrame=ContactFrame  SenseNormalForce=off  SenseNormalForceMagnitude=off  SenseNormalTorque=off  SenseFrictionalForce=off  SenseFrictionalForceMagnitude=off  SenseFrictionalTorque=off  SenseTotalForce=off  SenseTotalTorque=off  SenseContactBaseRotation=off  SenseContactBaseTranslation=off  SenseContactFollowerRotation=off  SenseContactFollowerTranslation=off  ZeroCrossDetectContactStartAndEnd=off
  Spherical Solid{,1..5} (6 alike) : sm_lib/Body Elements/Spherical Solid  SphereRadius=foot_r  SphereRadiusUnits=m  ExportEntireGeometry=on  InertiaType=CalculateFromGeometry  BasedOnType=Density  Density=1000  DensityUnits=kg/m^3  Mass=1  MassUnits=kg  CenterOfMass=[0 0 0]  CenterOfMassUnits=m  MomentsOfInertia=[1 1 1]  MomentsOfInertiaUnits=kg*m^2  ProductsOfInertia=[0 0 0]  ProductsOfInertiaUnits=kg*m^2  GraphicType=FromGeometry  MarkerShape=Sphere  MarkerSize=10  GraphicVisPropType=SimpleVisualProperties  GraphicDiffuseColor=[1 0.5 0.5]  GraphicOpacity=1  GraphicSpecularColor=[0.5 0.5 0.5 1.0]  GraphicAmbientColor=[0.15 0.15 0.15 1.0]  GraphicEmissiveColor=[0.0 0.0 0.0 1.0]  GraphicShininess=75  DoExposeReferenceFrame=on  SerializedFrames=<Frames/>
  Subsystem : Subsystem
  Subsystem1 : Subsystem
  Subsystem2 : Subsystem
  Subsystem3 : Subsystem
  Subsystem4 : Subsystem
  Subsystem5 : Subsystem
  Subtract : Sum  Inputs=+-
  Sum{,1..7} (8 alike) : Sum  Inputs=|++
  To Workspace : ToWorkspace  VariableName=torque_estim  SaveFormat=Timeseries  SampleTime=-1
  To Workspace1 : ToWorkspace  VariableName=torque_sens  SaveFormat=Timeseries  SampleTime=-1
  To Workspace10 : ToWorkspace  VariableName=c_lf  SaveFormat=Timeseries  SampleTime=-1
  To Workspace11 : ToWorkspace  VariableName=c_lm  SaveFormat=Timeseries  SampleTime=-1
  To Workspace12 : ToWorkspace  VariableName=c_lr  SaveFormat=Timeseries  SampleTime=-1
  To Workspace13 : ToWorkspace  VariableName=c_rf  SaveFormat=Timeseries  SampleTime=-1
  To Workspace14 : ToWorkspace  VariableName=c_rm  SaveFormat=Timeseries  SampleTime=-1
  To Workspace15 : ToWorkspace  VariableName=c_rr  SaveFormat=Timeseries  SampleTime=-1
  To Workspace2 : ToWorkspace  Commented=on  VariableName=Fsum  SaveFormat=Timeseries  SampleTime=-1
  To Workspace3 : ToWorkspace  VariableName=Fleg  SaveFormat=Timeseries  SampleTime=-1
  To Workspace4 : ToWorkspace  VariableName=z_lf  SaveFormat=Timeseries  SampleTime=-1
  To Workspace5 : ToWorkspace  VariableName=z_lm  SaveFormat=Timeseries  SampleTime=-1
  To Workspace6 : ToWorkspace  VariableName=z_lr  SaveFormat=Timeseries  SampleTime=-1
  To Workspace7 : ToWorkspace  VariableName=z_rf  SaveFormat=Timeseries  SampleTime=-1
  To Workspace8 : ToWorkspace  VariableName=z_rm  SaveFormat=Timeseries  SampleTime=-1
  To Workspace9 : ToWorkspace  VariableName=z_rr  SaveFormat=Timeseries  SampleTime=-1
  Transform Sensor : sm_lib/Frames and Transforms/Transform Sensor  MeasurementFrame=World  RotationSequence=ZYX  SenseAngle=off  SenseAxis=off  SenseQ=off  SenseR=off  SenseRotationSequence=on  SenseOmegaX=off  SenseOmegaY=off  SenseOmegaZ=off  SenseOmega=off  SenseQDot=off  SenseRDot=off  SenseRotationSequenceDot=off  SenseAlphaX=off  SenseAlphaY=off  SenseAlphaZ=off  SenseAlpha=off  SenseQDDot=off  SenseRDDot=off  SenseX=off  SenseY=off  SenseZ=off  SenseXYZ=on  SenseRad=off  SenseAzim=off  SenseDist=off  SenseInc=off  SenseXDot=off  SenseYDot=off  SenseZDot=off  SenseXYZDot=on  SenseRadDot=off  SenseAzimDot=off  SenseDistDot=off  SenseIncDot=off  SenseXDDot=off  SenseYDDot=off  SenseZDDot=off  SenseXYZDDot=off  SenseRadDDot=off  SenseAzimDDot=off  SenseDistDDot=off  SenseIncDDot=off
  Unit Delay{,1..5} (6 alike) : UnitDelay  SampleTime=-1  HasFrameUpgradeWarning=on
  Unit Delay6 : UnitDelay  SampleTime=0.001  HasFrameUpgradeWarning=on
  World : sm_lib/Frames and Transforms/World Frame
  X : Scope
      settings: ActiveDisplayYMinimum=-0.037357622523365976  ActiveDisplayYMaximum=0.0403053454057154  DataLoggingVariableName=ScopeData14
  Y : Scope
      settings: ActiveDisplayYMinimum=-0.25922967950892895  ActiveDisplayYMaximum=0.030350783325473713  DataLoggingVariableName=ScopeData13
  Z : Scope
      settings: ActiveDisplayYMinimum=-0.017279945118288426  ActiveDisplayYMaximum=0.014307521698995334  DataLoggingVariableName=ScopeData12
  base_link : Subsystem
  c1_lf : Subsystem
  c1_lm : Subsystem
  c1_lr : Subsystem
  c1_rf : Subsystem
  c1_rm : Subsystem
  c1_rr : Subsystem
  c2_lf : Subsystem
  c2_lm : Subsystem
  c2_lr : Subsystem
  c2_rf : Subsystem
  c2_rm : Subsystem
  c2_rr : Subsystem
  j_c1_lf : sm_lib/Joints/Revolute Joint  JointMode=Normal  CompositeWrenchDir=FollowerOnBase  CompositeWrenchFrame=BaseFrame  SenseConstraintForce=off  SenseConstraintTorque=off  SenseTotalForce=off  SenseTotalTorque=off  PositionTargetSpecify=off  PositionTargetPriority=High  PositionTargetValue=0  PositionTargetValueUnits=deg  VelocityTargetSpecify=off  VelocityTargetPriority=High  VelocityTargetValue=0  VelocityTargetValueUnits=deg/s  EquilibriumPosition=0  EquilibriumPositionUnits=deg  SpringStiffness=0  SpringStiffnessUnits=N*m/deg  DampingCoefficient=0  DampingCoefficientUnits=kg*m^2/(rad*s)  LowerLimitSpecify=on  LowerLimitBound=-2.6179939  LowerLimitBoundUnits=rad  LowerLimitStiffness=1e4  LowerLimitStiffnessUnits=N*m/deg  LowerLimitDamping=10  LowerLimitDampingUnits=N*m/(deg/s)  LowerLimitTransitionRegionWidth=0.1  LowerLimitTransitionRegionWidthUnits=deg  UpperLimitSpecify=on  UpperLimitBound=2.6179939  UpperLimitBoundUnits=rad  UpperLimitStiffness=1e4  UpperLimitStiffnessUnits=N*m/deg  UpperLimitDamping=10  UpperLimitDampingUnits=N*m/(deg/s)  UpperLimitTransitionRegionWidth=0.1  UpperLimitTransitionRegionWidthUnits=deg  TorqueActuationMode=ComputedTorque  MotionActuationMode=InputMotion  SensePosition=on  SenseVelocity=on  SenseAcceleration=on  SenseTorqueForce=on  SenseLowerLimitTorqueForce=off  SenseUpperLimitTorqueForce=off
  j_c1_lm : sm_lib/Joints/Revolute Joint  JointMode=Normal  CompositeWrenchDir=FollowerOnBase  CompositeWrenchFrame=BaseFrame  SenseConstraintForce=off  SenseConstraintTorque=off  SenseTotalForce=off  SenseTotalTorque=off  PositionTargetSpecify=off  PositionTargetPriority=High  PositionTargetValue=0  PositionTargetValueUnits=deg  VelocityTargetSpecify=off  VelocityTargetPriority=High  VelocityTargetValue=0  VelocityTargetValueUnits=deg/s  EquilibriumPosition=0  EquilibriumPositionUnits=deg  SpringStiffness=0  SpringStiffnessUnits=N*m/deg  DampingCoefficient=0  DampingCoefficientUnits=kg*m^2/(rad*s)  LowerLimitSpecify=on  LowerLimitBound=-2.6179939  LowerLimitBoundUnits=rad  LowerLimitStiffness=1e4  LowerLimitStiffnessUnits=N*m/deg  LowerLimitDamping=10  LowerLimitDampingUnits=N*m/(deg/s)  LowerLimitTransitionRegionWidth=0.1  LowerLimitTransitionRegionWidthUnits=deg  UpperLimitSpecify=on  UpperLimitBound=2.6179939  UpperLimitBoundUnits=rad  UpperLimitStiffness=1e4  UpperLimitStiffnessUnits=N*m/deg  UpperLimitDamping=10  UpperLimitDampingUnits=N*m/(deg/s)  UpperLimitTransitionRegionWidth=0.1  UpperLimitTransitionRegionWidthUnits=deg  TorqueActuationMode=ComputedTorque  MotionActuationMode=InputMotion  SensePosition=on  SenseVelocity=on  SenseAcceleration=on  SenseTorqueForce=on  SenseLowerLimitTorqueForce=off  SenseUpperLimitTorqueForce=off
  j_c1_lr : sm_lib/Joints/Revolute Joint  JointMode=Normal  CompositeWrenchDir=FollowerOnBase  CompositeWrenchFrame=BaseFrame  SenseConstraintForce=off  SenseConstraintTorque=off  SenseTotalForce=off  SenseTotalTorque=off  PositionTargetSpecify=off  PositionTargetPriority=High  PositionTargetValue=0  PositionTargetValueUnits=deg  VelocityTargetSpecify=off  VelocityTargetPriority=High  VelocityTargetValue=0  VelocityTargetValueUnits=deg/s  EquilibriumPosition=0  EquilibriumPositionUnits=deg  SpringStiffness=0  SpringStiffnessUnits=N*m/deg  DampingCoefficient=0  DampingCoefficientUnits=kg*m^2/(rad*s)  LowerLimitSpecify=on  LowerLimitBound=-2.6179939  LowerLimitBoundUnits=rad  LowerLimitStiffness=1e4  LowerLimitStiffnessUnits=N*m/deg  LowerLimitDamping=10  LowerLimitDampingUnits=N*m/(deg/s)  LowerLimitTransitionRegionWidth=0.1  LowerLimitTransitionRegionWidthUnits=deg  UpperLimitSpecify=on  UpperLimitBound=2.6179939  UpperLimitBoundUnits=rad  UpperLimitStiffness=1e4  UpperLimitStiffnessUnits=N*m/deg  UpperLimitDamping=10  UpperLimitDampingUnits=N*m/(deg/s)  UpperLimitTransitionRegionWidth=0.1  UpperLimitTransitionRegionWidthUnits=deg  TorqueActuationMode=ComputedTorque  MotionActuationMode=InputMotion  SensePosition=on  SenseVelocity=on  SenseAcceleration=on  SenseTorqueForce=on  SenseLowerLimitTorqueForce=off  SenseUpperLimitTorqueForce=off
  j_c1_rf : sm_lib/Joints/Revolute Joint  JointMode=Normal  CompositeWrenchDir=FollowerOnBase  CompositeWrenchFrame=BaseFrame  SenseConstraintForce=off  SenseConstraintTorque=off  SenseTotalForce=off  SenseTotalTorque=off  PositionTargetSpecify=off  PositionTargetPriority=High  PositionTargetValue=0  PositionTargetValueUnits=deg  VelocityTargetSpecify=off  VelocityTargetPriority=High  VelocityTargetValue=0  VelocityTargetValueUnits=deg/s  EquilibriumPosition=0  EquilibriumPositionUnits=deg  SpringStiffness=0  SpringStiffnessUnits=N*m/deg  DampingCoefficient=0  DampingCoefficientUnits=kg*m^2/(rad*s)  LowerLimitSpecify=on  LowerLimitBound=-2.6179939  LowerLimitBoundUnits=rad  LowerLimitStiffness=1e4  LowerLimitStiffnessUnits=N*m/deg  LowerLimitDamping=10  LowerLimitDampingUnits=N*m/(deg/s)  LowerLimitTransitionRegionWidth=0.1  LowerLimitTransitionRegionWidthUnits=deg  UpperLimitSpecify=on  UpperLimitBound=2.6179939  UpperLimitBoundUnits=rad  UpperLimitStiffness=1e4  UpperLimitStiffnessUnits=N*m/deg  UpperLimitDamping=10  UpperLimitDampingUnits=N*m/(deg/s)  UpperLimitTransitionRegionWidth=0.1  UpperLimitTransitionRegionWidthUnits=deg  TorqueActuationMode=ComputedTorque  MotionActuationMode=InputMotion  SensePosition=on  SenseVelocity=on  SenseAcceleration=on  SenseTorqueForce=on  SenseLowerLimitTorqueForce=off  SenseUpperLimitTorqueForce=off
  j_c1_rm : sm_lib/Joints/Revolute Joint  JointMode=Normal  CompositeWrenchDir=FollowerOnBase  CompositeWrenchFrame=BaseFrame  SenseConstraintForce=off  SenseConstraintTorque=off  SenseTotalForce=off  SenseTotalTorque=off  PositionTargetSpecify=off  PositionTargetPriority=High  PositionTargetValue=0  PositionTargetValueUnits=deg  VelocityTargetSpecify=off  VelocityTargetPriority=High  VelocityTargetValue=0  VelocityTargetValueUnits=deg/s  EquilibriumPosition=0  EquilibriumPositionUnits=deg  SpringStiffness=0  SpringStiffnessUnits=N*m/deg  DampingCoefficient=0  DampingCoefficientUnits=kg*m^2/(rad*s)  LowerLimitSpecify=on  LowerLimitBound=-2.6179939  LowerLimitBoundUnits=rad  LowerLimitStiffness=1e4  LowerLimitStiffnessUnits=N*m/deg  LowerLimitDamping=10  LowerLimitDampingUnits=N*m/(deg/s)  LowerLimitTransitionRegionWidth=0.1  LowerLimitTransitionRegionWidthUnits=deg  UpperLimitSpecify=on  UpperLimitBound=2.6179939  UpperLimitBoundUnits=rad  UpperLimitStiffness=1e4  UpperLimitStiffnessUnits=N*m/deg  UpperLimitDamping=10  UpperLimitDampingUnits=N*m/(deg/s)  UpperLimitTransitionRegionWidth=0.1  UpperLimitTransitionRegionWidthUnits=deg  TorqueActuationMode=ComputedTorque  MotionActuationMode=InputMotion  SensePosition=on  SenseVelocity=on  SenseAcceleration=on  SenseTorqueForce=on  SenseLowerLimitTorqueForce=off  SenseUpperLimitTorqueForce=off
  j_c1_rr : sm_lib/Joints/Revolute Joint  JointMode=Normal  CompositeWrenchDir=FollowerOnBase  CompositeWrenchFrame=BaseFrame  SenseConstraintForce=off  SenseConstraintTorque=off  SenseTotalForce=off  SenseTotalTorque=off  PositionTargetSpecify=off  PositionTargetPriority=High  PositionTargetValue=0  PositionTargetValueUnits=deg  VelocityTargetSpecify=off  VelocityTargetPriority=High  VelocityTargetValue=0  VelocityTargetValueUnits=deg/s  EquilibriumPosition=0  EquilibriumPositionUnits=deg  SpringStiffness=0  SpringStiffnessUnits=N*m/deg  DampingCoefficient=0  DampingCoefficientUnits=kg*m^2/(rad*s)  LowerLimitSpecify=on  LowerLimitBound=-2.6179939  LowerLimitBoundUnits=rad  LowerLimitStiffness=1e4  LowerLimitStiffnessUnits=N*m/deg  LowerLimitDamping=10  LowerLimitDampingUnits=N*m/(deg/s)  LowerLimitTransitionRegionWidth=0.1  LowerLimitTransitionRegionWidthUnits=deg  UpperLimitSpecify=on  UpperLimitBound=2.6179939  UpperLimitBoundUnits=rad  UpperLimitStiffness=1e4  UpperLimitStiffnessUnits=N*m/deg  UpperLimitDamping=10  UpperLimitDampingUnits=N*m/(deg/s)  UpperLimitTransitionRegionWidth=0.1  UpperLimitTransitionRegionWidthUnits=deg  TorqueActuationMode=ComputedTorque  MotionActuationMode=InputMotion  SensePosition=on  SenseVelocity=on  SenseAcceleration=on  SenseTorqueForce=on  SenseLowerLimitTorqueForce=off  SenseUpperLimitTorqueForce=off
  j_c2_lf : sm_lib/Joints/Weld Joint  JointMode=Normal  CompositeWrenchDir=FollowerOnBase  CompositeWrenchFrame=BaseFrame  SenseConstraintForce=off  SenseConstraintTorque=off  SenseTotalForce=off  SenseTotalTorque=off
  j_c2_lm : sm_lib/Joints/Weld Joint  JointMode=Normal  CompositeWrenchDir=FollowerOnBase  CompositeWrenchFrame=BaseFrame  SenseConstraintForce=off  SenseConstraintTorque=off  SenseTotalForce=off  SenseTotalTorque=off
  j_c2_lr : sm_lib/Joints/Weld Joint  JointMode=Normal  CompositeWrenchDir=FollowerOnBase  CompositeWrenchFrame=BaseFrame  SenseConstraintForce=off  SenseConstraintTorque=off  SenseTotalForce=off  SenseTotalTorque=off
  j_c2_rf : sm_lib/Joints/Weld Joint  JointMode=Normal  CompositeWrenchDir=FollowerOnBase  CompositeWrenchFrame=BaseFrame  SenseConstraintForce=off  SenseConstraintTorque=off  SenseTotalForce=off  SenseTotalTorque=off
  j_c2_rm : sm_lib/Joints/Weld Joint  JointMode=Normal  CompositeWrenchDir=FollowerOnBase  CompositeWrenchFrame=BaseFrame  SenseConstraintForce=off  SenseConstraintTorque=off  SenseTotalForce=off  SenseTotalTorque=off
  j_c2_rr : sm_lib/Joints/Weld Joint  JointMode=Normal  CompositeWrenchDir=FollowerOnBase  CompositeWrenchFrame=BaseFrame  SenseConstraintForce=off  SenseConstraintTorque=off  SenseTotalForce=off  SenseTotalTorque=off
  j_phantomx_attachment : sm_lib/Joints/Weld Joint  JointMode=Normal  CompositeWrenchDir=FollowerOnBase  CompositeWrenchFrame=BaseFrame  SenseConstraintForce=off  SenseConstraintTorque=off  SenseTotalForce=off  SenseTotalTorque=off
  j_thigh_lf : sm_lib/Joints/Revolute Joint  JointMode=Normal  CompositeWrenchDir=FollowerOnBase  CompositeWrenchFrame=BaseFrame  SenseConstraintForce=off  SenseConstraintTorque=off  SenseTotalForce=off  SenseTotalTorque=off  PositionTargetSpecify=off  PositionTargetPriority=High  PositionTargetValue=0  PositionTargetValueUnits=deg  VelocityTargetSpecify=off  VelocityTargetPriority=High  VelocityTargetValue=0  VelocityTargetValueUnits=deg/s  EquilibriumPosition=0  EquilibriumPositionUnits=deg  SpringStiffness=0  SpringStiffnessUnits=N*m/deg  DampingCoefficient=0  DampingCoefficientUnits=kg*m^2/(rad*s)  LowerLimitSpecify=on  LowerLimitBound=-2.6179939  LowerLimitBoundUnits=rad  LowerLimitStiffness=1e4  LowerLimitStiffnessUnits=N*m/deg  LowerLimitDamping=10  LowerLimitDampingUnits=N*m/(deg/s)  LowerLimitTransitionRegionWidth=0.1  LowerLimitTransitionRegionWidthUnits=deg  UpperLimitSpecify=on  UpperLimitBound=2.6179939  UpperLimitBoundUnits=rad  UpperLimitStiffness=1e4  UpperLimitStiffnessUnits=N*m/deg  UpperLimitDamping=10  UpperLimitDampingUnits=N*m/(deg/s)  UpperLimitTransitionRegionWidth=0.1  UpperLimitTransitionRegionWidthUnits=deg  TorqueActuationMode=ComputedTorque  MotionActuationMode=InputMotion  SensePosition=on  SenseVelocity=on  SenseAcceleration=on  SenseTorqueForce=on  SenseLowerLimitTorqueForce=off  SenseUpperLimitTorqueForce=off
  j_thigh_lm : sm_lib/Joints/Revolute Joint  JointMode=Normal  CompositeWrenchDir=FollowerOnBase  CompositeWrenchFrame=BaseFrame  SenseConstraintForce=off  SenseConstraintTorque=off  SenseTotalForce=off  SenseTotalTorque=off  PositionTargetSpecify=off  PositionTargetPriority=High  PositionTargetValue=0  PositionTargetValueUnits=deg  VelocityTargetSpecify=off  VelocityTargetPriority=High  VelocityTargetValue=0  VelocityTargetValueUnits=deg/s  EquilibriumPosition=0  EquilibriumPositionUnits=deg  SpringStiffness=0  SpringStiffnessUnits=N*m/deg  DampingCoefficient=0  DampingCoefficientUnits=kg*m^2/(rad*s)  LowerLimitSpecify=on  LowerLimitBound=-2.6179939  LowerLimitBoundUnits=rad  LowerLimitStiffness=1e4  LowerLimitStiffnessUnits=N*m/deg  LowerLimitDamping=10  LowerLimitDampingUnits=N*m/(deg/s)  LowerLimitTransitionRegionWidth=0.1  LowerLimitTransitionRegionWidthUnits=deg  UpperLimitSpecify=on  UpperLimitBound=2.6179939  UpperLimitBoundUnits=rad  UpperLimitStiffness=1e4  UpperLimitStiffnessUnits=N*m/deg  UpperLimitDamping=10  UpperLimitDampingUnits=N*m/(deg/s)  UpperLimitTransitionRegionWidth=0.1  UpperLimitTransitionRegionWidthUnits=deg  TorqueActuationMode=ComputedTorque  MotionActuationMode=InputMotion  SensePosition=on  SenseVelocity=on  SenseAcceleration=on  SenseTorqueForce=on  SenseLowerLimitTorqueForce=off  SenseUpperLimitTorqueForce=off
  j_thigh_lr : sm_lib/Joints/Revolute Joint  JointMode=Normal  CompositeWrenchDir=FollowerOnBase  CompositeWrenchFrame=BaseFrame  SenseConstraintForce=off  SenseConstraintTorque=off  SenseTotalForce=off  SenseTotalTorque=off  PositionTargetSpecify=off  PositionTargetPriority=High  PositionTargetValue=0  PositionTargetValueUnits=deg  VelocityTargetSpecify=off  VelocityTargetPriority=High  VelocityTargetValue=0  VelocityTargetValueUnits=deg/s  EquilibriumPosition=0  EquilibriumPositionUnits=deg  SpringStiffness=0  SpringStiffnessUnits=N*m/deg  DampingCoefficient=0  DampingCoefficientUnits=kg*m^2/(rad*s)  LowerLimitSpecify=on  LowerLimitBound=-2.6179939  LowerLimitBoundUnits=rad  LowerLimitStiffness=1e4  LowerLimitStiffnessUnits=N*m/deg  LowerLimitDamping=10  LowerLimitDampingUnits=N*m/(deg/s)  LowerLimitTransitionRegionWidth=0.1  LowerLimitTransitionRegionWidthUnits=deg  UpperLimitSpecify=on  UpperLimitBound=2.6179939  UpperLimitBoundUnits=rad  UpperLimitStiffness=1e4  UpperLimitStiffnessUnits=N*m/deg  UpperLimitDamping=10  UpperLimitDampingUnits=N*m/(deg/s)  UpperLimitTransitionRegionWidth=0.1  UpperLimitTransitionRegionWidthUnits=deg  TorqueActuationMode=ComputedTorque  MotionActuationMode=InputMotion  SensePosition=on  SenseVelocity=on  SenseAcceleration=on  SenseTorqueForce=on  SenseLowerLimitTorqueForce=off  SenseUpperLimitTorqueForce=off
  j_thigh_rf : sm_lib/Joints/Revolute Joint  JointMode=Normal  CompositeWrenchDir=FollowerOnBase  CompositeWrenchFrame=BaseFrame  SenseConstraintForce=off  SenseConstraintTorque=off  SenseTotalForce=off  SenseTotalTorque=off  PositionTargetSpecify=off  PositionTargetPriority=High  PositionTargetValue=0  PositionTargetValueUnits=deg  VelocityTargetSpecify=off  VelocityTargetPriority=High  VelocityTargetValue=0  VelocityTargetValueUnits=deg/s  EquilibriumPosition=0  EquilibriumPositionUnits=deg  SpringStiffness=0  SpringStiffnessUnits=N*m/deg  DampingCoefficient=0  DampingCoefficientUnits=kg*m^2/(rad*s)  LowerLimitSpecify=on  LowerLimitBound=-2.6179939  LowerLimitBoundUnits=rad  LowerLimitStiffness=1e4  LowerLimitStiffnessUnits=N*m/deg  LowerLimitDamping=10  LowerLimitDampingUnits=N*m/(deg/s)  LowerLimitTransitionRegionWidth=0.1  LowerLimitTransitionRegionWidthUnits=deg  UpperLimitSpecify=on  UpperLimitBound=2.6179939  UpperLimitBoundUnits=rad  UpperLimitStiffness=1e4  UpperLimitStiffnessUnits=N*m/deg  UpperLimitDamping=10  UpperLimitDampingUnits=N*m/(deg/s)  UpperLimitTransitionRegionWidth=0.1  UpperLimitTransitionRegionWidthUnits=deg  TorqueActuationMode=ComputedTorque  MotionActuationMode=InputMotion  SensePosition=on  SenseVelocity=on  SenseAcceleration=on  SenseTorqueForce=on  SenseLowerLimitTorqueForce=off  SenseUpperLimitTorqueForce=off
  j_thigh_rm : sm_lib/Joints/Revolute Joint  JointMode=Normal  CompositeWrenchDir=FollowerOnBase  CompositeWrenchFrame=BaseFrame  SenseConstraintForce=off  SenseConstraintTorque=off  SenseTotalForce=off  SenseTotalTorque=off  PositionTargetSpecify=off  PositionTargetPriority=High  PositionTargetValue=0  PositionTargetValueUnits=deg  VelocityTargetSpecify=off  VelocityTargetPriority=High  VelocityTargetValue=0  VelocityTargetValueUnits=deg/s  EquilibriumPosition=0  EquilibriumPositionUnits=deg  SpringStiffness=0  SpringStiffnessUnits=N*m/deg  DampingCoefficient=0  DampingCoefficientUnits=kg*m^2/(rad*s)  LowerLimitSpecify=on  LowerLimitBound=-2.6179939  LowerLimitBoundUnits=rad  LowerLimitStiffness=1e4  LowerLimitStiffnessUnits=N*m/deg  LowerLimitDamping=10  LowerLimitDampingUnits=N*m/(deg/s)  LowerLimitTransitionRegionWidth=0.1  LowerLimitTransitionRegionWidthUnits=deg  UpperLimitSpecify=on  UpperLimitBound=2.6179939  UpperLimitBoundUnits=rad  UpperLimitStiffness=1e4  UpperLimitStiffnessUnits=N*m/deg  UpperLimitDamping=10  UpperLimitDampingUnits=N*m/(deg/s)  UpperLimitTransitionRegionWidth=0.1  UpperLimitTransitionRegionWidthUnits=deg  TorqueActuationMode=ComputedTorque  MotionActuationMode=InputMotion  SensePosition=on  SenseVelocity=on  SenseAcceleration=on  SenseTorqueForce=on  SenseLowerLimitTorqueForce=off  SenseUpperLimitTorqueForce=off
  j_thigh_rr : sm_lib/Joints/Revolute Joint  JointMode=Normal  CompositeWrenchDir=FollowerOnBase  CompositeWrenchFrame=BaseFrame  SenseConstraintForce=off  SenseConstraintTorque=off  SenseTotalForce=off  SenseTotalTorque=off  PositionTargetSpecify=off  PositionTargetPriority=High  PositionTargetValue=0  PositionTargetValueUnits=deg  VelocityTargetSpecify=off  VelocityTargetPriority=High  VelocityTargetValue=0  VelocityTargetValueUnits=deg/s  EquilibriumPosition=0  EquilibriumPositionUnits=deg  SpringStiffness=0  SpringStiffnessUnits=N*m/deg  DampingCoefficient=0  DampingCoefficientUnits=kg*m^2/(rad*s)  LowerLimitSpecify=on  LowerLimitBound=-2.6179939  LowerLimitBoundUnits=rad  LowerLimitStiffness=1e4  LowerLimitStiffnessUnits=N*m/deg  LowerLimitDamping=10  LowerLimitDampingUnits=N*m/(deg/s)  LowerLimitTransitionRegionWidth=0.1  LowerLimitTransitionRegionWidthUnits=deg  UpperLimitSpecify=on  UpperLimitBound=2.6179939  UpperLimitBoundUnits=rad  UpperLimitStiffness=1e4  UpperLimitStiffnessUnits=N*m/deg  UpperLimitDamping=10  UpperLimitDampingUnits=N*m/(deg/s)  UpperLimitTransitionRegionWidth=0.1  UpperLimitTransitionRegionWidthUnits=deg  TorqueActuationMode=ComputedTorque  MotionActuationMode=InputMotion  SensePosition=on  SenseVelocity=on  SenseAcceleration=on  SenseTorqueForce=on  SenseLowerLimitTorqueForce=off  SenseUpperLimitTorqueForce=off
  j_tibia_lf : sm_lib/Joints/Revolute Joint  JointMode=Normal  CompositeWrenchDir=FollowerOnBase  CompositeWrenchFrame=BaseFrame  SenseConstraintForce=off  SenseConstraintTorque=off  SenseTotalForce=off  SenseTotalTorque=off  PositionTargetSpecify=off  PositionTargetPriority=High  PositionTargetValue=0  PositionTargetValueUnits=deg  VelocityTargetSpecify=off  VelocityTargetPriority=High  VelocityTargetValue=0  VelocityTargetValueUnits=deg/s  EquilibriumPosition=0  EquilibriumPositionUnits=deg  SpringStiffness=0  SpringStiffnessUnits=N*m/deg  DampingCoefficient=0  DampingCoefficientUnits=kg*m^2/(rad*s)  LowerLimitSpecify=on  LowerLimitBound=-2.6179939  LowerLimitBoundUnits=rad  LowerLimitStiffness=1e4  LowerLimitStiffnessUnits=N*m/deg  LowerLimitDamping=10  LowerLimitDampingUnits=N*m/(deg/s)  LowerLimitTransitionRegionWidth=0.1  LowerLimitTransitionRegionWidthUnits=deg  UpperLimitSpecify=on  UpperLimitBound=2.6179939  UpperLimitBoundUnits=rad  UpperLimitStiffness=1e4  UpperLimitStiffnessUnits=N*m/deg  UpperLimitDamping=10  UpperLimitDampingUnits=N*m/(deg/s)  UpperLimitTransitionRegionWidth=0.1  UpperLimitTransitionRegionWidthUnits=deg  TorqueActuationMode=ComputedTorque  MotionActuationMode=InputMotion  SensePosition=on  SenseVelocity=on  SenseAcceleration=on  SenseTorqueForce=on  SenseLowerLimitTorqueForce=off  SenseUpperLimitTorqueForce=off
  j_tibia_lm : sm_lib/Joints/Revolute Joint  JointMode=Normal  CompositeWrenchDir=FollowerOnBase  CompositeWrenchFrame=BaseFrame  SenseConstraintForce=off  SenseConstraintTorque=off  SenseTotalForce=off  SenseTotalTorque=off  PositionTargetSpecify=off  PositionTargetPriority=High  PositionTargetValue=0  PositionTargetValueUnits=deg  VelocityTargetSpecify=off  VelocityTargetPriority=High  VelocityTargetValue=0  VelocityTargetValueUnits=deg/s  EquilibriumPosition=0  EquilibriumPositionUnits=deg  SpringStiffness=0  SpringStiffnessUnits=N*m/deg  DampingCoefficient=0  DampingCoefficientUnits=kg*m^2/(rad*s)  LowerLimitSpecify=on  LowerLimitBound=-2.6179939  LowerLimitBoundUnits=rad  LowerLimitStiffness=1e4  LowerLimitStiffnessUnits=N*m/deg  LowerLimitDamping=10  LowerLimitDampingUnits=N*m/(deg/s)  LowerLimitTransitionRegionWidth=0.1  LowerLimitTransitionRegionWidthUnits=deg  UpperLimitSpecify=on  UpperLimitBound=2.6179939  UpperLimitBoundUnits=rad  UpperLimitStiffness=1e4  UpperLimitStiffnessUnits=N*m/deg  UpperLimitDamping=10  UpperLimitDampingUnits=N*m/(deg/s)  UpperLimitTransitionRegionWidth=0.1  UpperLimitTransitionRegionWidthUnits=deg  TorqueActuationMode=ComputedTorque  MotionActuationMode=InputMotion  SensePosition=on  SenseVelocity=on  SenseAcceleration=on  SenseTorqueForce=on  SenseLowerLimitTorqueForce=off  SenseUpperLimitTorqueForce=off
  j_tibia_lr : sm_lib/Joints/Revolute Joint  JointMode=Normal  CompositeWrenchDir=FollowerOnBase  CompositeWrenchFrame=BaseFrame  SenseConstraintForce=off  SenseConstraintTorque=off  SenseTotalForce=off  SenseTotalTorque=off  PositionTargetSpecify=off  PositionTargetPriority=High  PositionTargetValue=0  PositionTargetValueUnits=deg  VelocityTargetSpecify=off  VelocityTargetPriority=High  VelocityTargetValue=0  VelocityTargetValueUnits=deg/s  EquilibriumPosition=0  EquilibriumPositionUnits=deg  SpringStiffness=0  SpringStiffnessUnits=N*m/deg  DampingCoefficient=0  DampingCoefficientUnits=kg*m^2/(rad*s)  LowerLimitSpecify=on  LowerLimitBound=-2.6179939  LowerLimitBoundUnits=rad  LowerLimitStiffness=1e4  LowerLimitStiffnessUnits=N*m/deg  LowerLimitDamping=10  LowerLimitDampingUnits=N*m/(deg/s)  LowerLimitTransitionRegionWidth=0.1  LowerLimitTransitionRegionWidthUnits=deg  UpperLimitSpecify=on  UpperLimitBound=2.6179939  UpperLimitBoundUnits=rad  UpperLimitStiffness=1e4  UpperLimitStiffnessUnits=N*m/deg  UpperLimitDamping=10  UpperLimitDampingUnits=N*m/(deg/s)  UpperLimitTransitionRegionWidth=0.1  UpperLimitTransitionRegionWidthUnits=deg  TorqueActuationMode=ComputedTorque  MotionActuationMode=InputMotion  SensePosition=on  SenseVelocity=on  SenseAcceleration=on  SenseTorqueForce=on  SenseLowerLimitTorqueForce=off  SenseUpperLimitTorqueForce=off
  j_tibia_rf : sm_lib/Joints/Revolute Joint  JointMode=Normal  CompositeWrenchDir=FollowerOnBase  CompositeWrenchFrame=BaseFrame  SenseConstraintForce=off  SenseConstraintTorque=off  SenseTotalForce=off  SenseTotalTorque=off  PositionTargetSpecify=off  PositionTargetPriority=High  PositionTargetValue=0  PositionTargetValueUnits=deg  VelocityTargetSpecify=off  VelocityTargetPriority=High  VelocityTargetValue=0  VelocityTargetValueUnits=deg/s  EquilibriumPosition=0  EquilibriumPositionUnits=deg  SpringStiffness=0  SpringStiffnessUnits=N*m/deg  DampingCoefficient=0  DampingCoefficientUnits=kg*m^2/(rad*s)  LowerLimitSpecify=on  LowerLimitBound=-2.6179939  LowerLimitBoundUnits=rad  LowerLimitStiffness=1e4  LowerLimitStiffnessUnits=N*m/deg  LowerLimitDamping=10  LowerLimitDampingUnits=N*m/(deg/s)  LowerLimitTransitionRegionWidth=0.1  LowerLimitTransitionRegionWidthUnits=deg  UpperLimitSpecify=on  UpperLimitBound=2.6179939  UpperLimitBoundUnits=rad  UpperLimitStiffness=1e4  UpperLimitStiffnessUnits=N*m/deg  UpperLimitDamping=10  UpperLimitDampingUnits=N*m/(deg/s)  UpperLimitTransitionRegionWidth=0.1  UpperLimitTransitionRegionWidthUnits=deg  TorqueActuationMode=ComputedTorque  MotionActuationMode=InputMotion  SensePosition=on  SenseVelocity=on  SenseAcceleration=on  SenseTorqueForce=on  SenseLowerLimitTorqueForce=off  SenseUpperLimitTorqueForce=off
  j_tibia_rm : sm_lib/Joints/Revolute Joint  JointMode=Normal  CompositeWrenchDir=FollowerOnBase  CompositeWrenchFrame=BaseFrame  SenseConstraintForce=off  SenseConstraintTorque=off  SenseTotalForce=off  SenseTotalTorque=off  PositionTargetSpecify=off  PositionTargetPriority=High  PositionTargetValue=0  PositionTargetValueUnits=deg  VelocityTargetSpecify=off  VelocityTargetPriority=High  VelocityTargetValue=0  VelocityTargetValueUnits=deg/s  EquilibriumPosition=0  EquilibriumPositionUnits=deg  SpringStiffness=0  SpringStiffnessUnits=N*m/deg  DampingCoefficient=0  DampingCoefficientUnits=kg*m^2/(rad*s)  LowerLimitSpecify=on  LowerLimitBound=-2.6179939  LowerLimitBoundUnits=rad  LowerLimitStiffness=1e4  LowerLimitStiffnessUnits=N*m/deg  LowerLimitDamping=10  LowerLimitDampingUnits=N*m/(deg/s)  LowerLimitTransitionRegionWidth=0.1  LowerLimitTransitionRegionWidthUnits=deg  UpperLimitSpecify=on  UpperLimitBound=2.6179939  UpperLimitBoundUnits=rad  UpperLimitStiffness=1e4  UpperLimitStiffnessUnits=N*m/deg  UpperLimitDamping=10  UpperLimitDampingUnits=N*m/(deg/s)  UpperLimitTransitionRegionWidth=0.1  UpperLimitTransitionRegionWidthUnits=deg  TorqueActuationMode=ComputedTorque  MotionActuationMode=InputMotion  SensePosition=on  SenseVelocity=on  SenseAcceleration=on  SenseTorqueForce=on  SenseLowerLimitTorqueForce=off  SenseUpperLimitTorqueForce=off
  j_tibia_rr : sm_lib/Joints/Revolute Joint  JointMode=Normal  CompositeWrenchDir=FollowerOnBase  CompositeWrenchFrame=BaseFrame  SenseConstraintForce=off  SenseConstraintTorque=off  SenseTotalForce=off  SenseTotalTorque=off  PositionTargetSpecify=off  PositionTargetPriority=High  PositionTargetValue=0  PositionTargetValueUnits=deg  VelocityTargetSpecify=off  VelocityTargetPriority=High  VelocityTargetValue=0  VelocityTargetValueUnits=deg/s  EquilibriumPosition=0  EquilibriumPositionUnits=deg  SpringStiffness=0  SpringStiffnessUnits=N*m/deg  DampingCoefficient=0  DampingCoefficientUnits=kg*m^2/(rad*s)  LowerLimitSpecify=on  LowerLimitBound=-2.6179939  LowerLimitBoundUnits=rad  LowerLimitStiffness=1e4  LowerLimitStiffnessUnits=N*m/deg  LowerLimitDamping=10  LowerLimitDampingUnits=N*m/(deg/s)  LowerLimitTransitionRegionWidth=0.1  LowerLimitTransitionRegionWidthUnits=deg  UpperLimitSpecify=on  UpperLimitBound=2.6179939  UpperLimitBoundUnits=rad  UpperLimitStiffness=1e4  UpperLimitStiffnessUnits=N*m/deg  UpperLimitDamping=10  UpperLimitDampingUnits=N*m/(deg/s)  UpperLimitTransitionRegionWidth=0.1  UpperLimitTransitionRegionWidthUnits=deg  TorqueActuationMode=ComputedTorque  MotionActuationMode=InputMotion  SensePosition=on  SenseVelocity=on  SenseAcceleration=on  SenseTorqueForce=on  SenseLowerLimitTorqueForce=off  SenseUpperLimitTorqueForce=off
  offset : Constant  Value=0
  positions : Scope
      settings: ActiveDisplayYMinimum=-0.39920679922920854  ActiveDisplayYMaximum=0.62338947283532586
  rotation sequence : Scope
      settings: ActiveDisplayYMinimum=-0.30159158006805792  ActiveDisplayYMaximum=0.065712171305191164  DataLoggingVariableName=ScopeData2
  thigh_lf : Subsystem
  thigh_lm : Subsystem
  thigh_lr : Subsystem
  thigh_rf : Subsystem
  thigh_rm : Subsystem
  thigh_rr : Subsystem
  tibia_lf : Subsystem
  tibia_lm : Subsystem
  tibia_lr : Subsystem
  tibia_rf : Subsystem
  tibia_rm : Subsystem
  tibia_rr : Subsystem
  velocities : Scope
      settings: ActiveDisplayYMinimum=-2.2914297070805834  ActiveDisplayYMaximum=0.912538212205687
  wires:
  PS-Simulink Converter3/1 -> [th_rr_q], Data Store Write1/1
  PS-Simulink Converter4/1 -> [t_rr_q], Data Store Write2/1
  PS-Simulink Converter7/1 -> [c_rm_q], Data Store Write3/1
  PS-Simulink Converter8/1 -> [th_rm_q], Data Store Write4/1
  PS-Simulink Converter9/1 -> Data Store Write5/1, [t_rm_q]
  PS-Simulink Converter5/1 -> [c_rf_q], Data Store Write6/1
  PS-Simulink Converter20/1 -> [th_rf_q], Data Store Write7/1
  PS-Simulink Converter6/1 -> Data Store Write8/1, [t_rf_q]
  PS-Simulink Converter11/1 -> [th_lr_q], Data Store Write10/1
  PS-Simulink Converter12/1 -> [t_lr_q], Data Store Write11/1
  PS-Simulink Converter10/1 -> [c_lr_q], Data Store Write9/1
  PS-Simulink Converter13/1 -> [c_lm_q], Data Store Write12/1
  PS-Simulink Converter14/1 -> [th_lm_q], Data Store Write13/1
  PS-Simulink Converter15/1 -> Data Store Write14/1, [t_lm_q]
  PS-Simulink Converter16/1 -> [c_lf_q], Data Store Write15/1
  PS-Simulink Converter17/1 -> [th_lf_q], Data Store Write16/1
  PS-Simulink Converter18/1 -> [t_lf_q], Data Store Write17/1
  PS-Simulink Converter1/1 -> rotation sequence/1, Demux8/1, Data Store Write18/1
  PS-Simulink Converter/1 -> [c_rr_q], Data Store Write/1
  [ref_joints] -> Display/1
  [ref_joints] -> Selector/1
  Selector/1 -> Simulink-PS Converter/1
  Selector1/1 -> Simulink-PS Converter1/1
  [ref_joints] -> Selector1/1
  Selector2/1 -> Simulink-PS Converter2/1
  Selector3/1 -> Simulink-PS Converter3/1
  [ref_joints] -> Selector3/1
  [ref_joints] -> Selector4/1
  Selector4/1 -> Simulink-PS Converter4/1
  [ref_joints] -> Selector5/1
  [ref_joints] -> Selector6/1
  [ref_joints] -> Selector7/1
  [ref_joints] -> Selector8/1
  Selector8/1 -> Simulink-PS Converter8/1
  Selector9/1 -> Simulink-PS Converter9/1
  [ref_joints] -> Selector9/1
  [ref_joints] -> Selector10/1
  Selector11/1 -> Simulink-PS Converter23/1
  [ref_joints] -> Selector11/1
  [ref_joints] -> Selector12/1
  Selector12/1 -> Simulink-PS Converter21/1
  Selector13/1 -> Simulink-PS Converter7/1
  [ref_joints] -> Selector13/1
  [ref_joints] -> Selector14/1
  Selector15/1 -> Simulink-PS Converter20/1
  [ref_joints] -> Selector15/1
  [ref_joints] -> Selector16/1
  Selector16/1 -> Simulink-PS Converter22/1
  Selector17/1 -> Simulink-PS Converter24/1
  [ref_joints] -> Selector17/1
  Selector5/1 -> Simulink-PS Converter18/1
  Selector6/1 -> Simulink-PS Converter5/1
  Selector7/1 -> Simulink-PS Converter6/1
  Selector10/1 -> Simulink-PS Converter25/1
  Selector14/1 -> Simulink-PS Converter19/1
  [ref_joints] -> Selector2/1
  PS-Simulink Converter19/1 -> positions/1
  PS-Simulink Converter2/1 -> velocities/1
  Sum/1 -> [ref_joints]
  Mux8/1 -> Sum/1
  offset/1 -> Sum/2
  RR/1(theta) -> Mux8/1
  RR/2(phi) -> Mux8/2
  RR/3(psi) -> Mux8/3
  MR/2(phi) -> Mux8/5
  MR/1(theta) -> Mux8/4
  MR/3(psi) -> Mux8/6
  FR/2(phi) -> Mux8/8
  FR/3(psi) -> Mux8/9
  RL/1(theta) -> Mux8/10
  ML/2(phi) -> Mux8/14
  ML/3(psi) -> Mux8/15
  FL/2(phi) -> Mux8/17
  RL/2(phi) -> Mux8/11
  RL/3(psi) -> Mux8/12
  ML/1(theta) -> Mux8/13
  Constant21/1 -> FR/5(alpha)
  Constant19/1 -> RR/5(alpha)
  Constant20/1 -> MR/5(alpha)
  Constant25/1 -> RL/5(alpha)
  Constant26/1 -> ML/5(alpha)
  Constant27/1 -> FL/5(alpha)
  FL/1(theta) -> Mux8/16
  FL/3(psi) -> Mux8/18
  FR/1(theta) -> Mux8/7
  Constant22/1 -> [RIGHT]
  [RIGHT] -> RR/4(side)
  [RIGHT] -> MR/4(side)
  [RIGHT] -> FR/4(side)
  Constant23/1 -> [LEFT]
  [LEFT] -> RL/4(side)
  [LEFT] -> ML/4(side)
  [LEFT] -> FL/4(side)
  Clock/1 -> MATLAB Function/1(t_in)
  Clock1/1 -> Add/1
  Constant28/1 -> Add/2
  MATLAB Function/1(x) -> [x1]
  [x2] -> RR/1(x)
  MATLAB Function/2(y) -> [y1]
  MATLAB Function/3(z) -> Scope7/1, [z1]
  MATLAB Function1/3(z) -> [z2]
  MATLAB Function1/2(y) -> [y2]
  MATLAB Function1/1(x) -> [x2]
  Add/1 -> MATLAB Function1/1(t_in)
  [y2] -> RR/2(y)
  [x1] -> MR/1(x)
  [y1] -> MR/2(y)
  [x2] -> FR/1(x)
  [y2] -> FR/2(y)
  [y1] -> RL/2(y)
  [x1] -> RL/1(x)
  [y2] -> ML/2(y)
  [x2] -> ML/1(x)
  [x1] -> FL/1(x)
  [y1] -> FL/2(y)
  Constant2/1 -> MATLAB Function/2(T)
  Constant3/1 -> MATLAB Function/3(S)
  Constant4/1 -> MATLAB Function/4(H)
  Constant5/1 -> MATLAB Function/5(z0)
  Constant9/1 -> MATLAB Function1/5(z0)
  Constant8/1 -> MATLAB Function1/4(H)
  Constant7/1 -> MATLAB Function1/3(S)
  Constant6/1 -> MATLAB Function1/2(T)
  Mux/1 -> Inverse Dynamics/1
  PS-Simulink Converter21/1 -> [c_rr_dq]
  PS-Simulink Converter22/1 -> [th_rr_dq]
  PS-Simulink Converter23/1 -> [t_rr_dq]
  PS-Simulink Converter24/1 -> [c_rr_ddq]
  PS-Simulink Converter25/1 -> [th_rr_ddq]
  PS-Simulink Converter26/1 -> [t_rr_ddq]
  Inverse Dynamics/1 -> To Workspace/1, Subtract/2, Demux/1
  Demux/1 -> Scope/1
  Demux/2 -> Scope/2
  Demux/3 -> Scope/3
  PS-Simulink Converter27/1 -> [c_rr_t]
  Mux3/1 -> To Workspace1/1, Subtract/1
  PS-Simulink Converter28/1 -> [th_rr_t]
  PS-Simulink Converter29/1 -> [t_rr_t]
  PS-Simulink Converter30/1 -> [c_rm_dq]
  PS-Simulink Converter31/1 -> [c_rm_ddq]
  PS-Simulink Converter32/1 -> [c_rm_t]
  PS-Simulink Converter33/1 -> [c_rf_dq]
  PS-Simulink Converter34/1 -> [c_rf_ddq]
  PS-Simulink Converter35/1 -> [c_rf_t]
  PS-Simulink Converter36/1 -> [c_lr_dq]
  PS-Simulink Converter37/1 -> [c_lr_ddq]
  PS-Simulink Converter38/1 -> [c_lr_t]
  PS-Simulink Converter39/1 -> [c_lm_dq]
  PS-Simulink Converter40/1 -> [c_lm_ddq]
  PS-Simulink Converter41/1 -> [c_lm_t]
  PS-Simulink Converter42/1 -> [c_lf_dq]
  PS-Simulink Converter43/1 -> [c_lf_ddq]
  PS-Simulink Converter44/1 -> [c_lf_t]
  PS-Simulink Converter45/1 -> [th_rm_dq]
  PS-Simulink Converter46/1 -> [th_rm_ddq]
  PS-Simulink Converter47/1 -> [th_rm_t]
  PS-Simulink Converter51/1 -> [th_lr_dq]
  PS-Simulink Converter53/1 -> [th_lr_t]
  PS-Simulink Converter48/1 -> [th_rf_dq]
  PS-Simulink Converter49/1 -> [th_rf_ddq]
  PS-Simulink Converter50/1 -> [th_rf_t]
  PS-Simulink Converter52/1 -> [th_lr_ddq]
  PS-Simulink Converter54/1 -> [th_lm_dq]
  PS-Simulink Converter55/1 -> [th_lm_ddq]
  PS-Simulink Converter56/1 -> [th_lm_t]
  PS-Simulink Converter57/1 -> [th_lf_dq]
  PS-Simulink Converter58/1 -> [th_lf_ddq]
  PS-Simulink Converter59/1 -> [th_lf_t]
  PS-Simulink Converter60/1 -> [t_rm_dq]
  PS-Simulink Converter61/1 -> [t_rm_ddq]
  PS-Simulink Converter62/1 -> [t_rm_t]
  PS-Simulink Converter63/1 -> [t_rf_dq]
  PS-Simulink Converter64/1 -> [t_rf_ddq]
  PS-Simulink Converter65/1 -> [t_rf_t]
  PS-Simulink Converter66/1 -> [t_lr_dq]
  PS-Simulink Converter67/1 -> [t_lr_ddq]
  PS-Simulink Converter68/1 -> [t_lr_t]
  PS-Simulink Converter69/1 -> [t_lm_dq]
  PS-Simulink Converter70/1 -> [t_lm_ddq]
  PS-Simulink Converter71/1 -> [t_lm_t]
  PS-Simulink Converter72/1 -> [t_lf_dq]
  PS-Simulink Converter73/1 -> [t_lf_ddq]
  PS-Simulink Converter74/1 -> [t_lf_t]
  [c_lf_q] -> Mux4/1
  [th_lf_q] -> Mux4/2
  [t_lf_q] -> Mux4/3
  Mux4/1 -> Mux/1
  [th_lm_q] -> Mux5/2
  [c_lm_q] -> Mux5/1
  Mux5/1 -> Mux/2
  [t_lm_q] -> Mux5/3
  [c_lr_q] -> Mux6/1
  [th_lr_q] -> Mux6/2
  [t_lr_q] -> Mux6/3
  Mux7/1 -> Mux/4
  [th_rf_q] -> Mux7/2
  [t_rf_q] -> Mux7/3
  [c_rf_q] -> Mux7/1
  [th_rm_q] -> Mux9/2
  [t_rm_q] -> Mux9/3
  Mux9/1 -> Mux/5
  [c_rm_q] -> Mux9/1
  [th_rr_q] -> Mux10/2
  [c_rr_q] -> Mux10/1
  [t_rr_q] -> Mux10/3
  Mux10/1 -> Mux/6
  Mux6/1 -> Mux/3
  [th_lr_dq] -> Mux14/2
  [c_lr_dq] -> Mux14/1
  [t_lf_dq] -> Mux12/3
  Mux13/1 -> Mux1/2
  Mux16/1 -> Mux1/5
  [t_rr_dq] -> Mux11/3
  [c_rr_dq] -> Mux11/1
  [th_rr_dq] -> Mux11/2
  [th_rm_dq] -> Mux16/2
  [c_rm_dq] -> Mux16/1
  [t_rm_dq] -> Mux16/3
  [t_rf_dq] -> Mux15/3
  [c_rf_dq] -> Mux15/1
  Mux15/1 -> Mux1/4
  [c_lm_dq] -> Mux13/1
  [t_lm_dq] -> Mux13/3
  Mux14/1 -> Mux1/3
  [th_lf_dq] -> Mux12/2
  [th_lm_dq] -> Mux13/2
  [c_lf_dq] -> Mux12/1
  [th_rf_dq] -> Mux15/2
  Mux12/1 -> Mux1/1
  Mux1/1 -> Inverse Dynamics/2
  [t_lr_dq] -> Mux14/3
  Mux11/1 -> Mux1/6
  [c_rf_ddq] -> Mux21/1
  [t_rf_ddq] -> Mux21/3
  Mux20/1 -> Mux2/3
  [t_lm_ddq] -> Mux19/3
  [c_lm_ddq] -> Mux19/1
  Mux21/1 -> Mux2/4
  [th_rr_ddq] -> Mux17/2
  [t_rm_ddq] -> Mux22/3
  [c_rm_ddq] -> Mux22/1
  [th_lr_ddq] -> Mux20/2
  [th_rm_ddq] -> Mux22/2
  [t_rr_ddq] -> Mux17/3
  [c_lr_ddq] -> Mux20/1
  Mux22/1 -> Mux2/5
  [t_lf_ddq] -> Mux18/3
  Mux19/1 -> Mux2/2
  [c_rr_ddq] -> Mux17/1
  Mux2/1 -> Inverse Dynamics/3
  [c_lf_ddq] -> Mux18/1
  Mux18/1 -> Mux2/1
  [th_lf_ddq] -> Mux18/2
  [th_rf_ddq] -> Mux21/2
  [th_lm_ddq] -> Mux19/2
  Mux17/1 -> Mux2/6
  [t_lr_ddq] -> Mux20/3
  [th_lr_t] -> Mux26/2
  [c_lr_t] -> Mux26/1
  [t_lf_t] -> Mux24/3
  Mux25/1 -> Mux3/2
  Mux28/1 -> Mux3/5
  [t_rr_t] -> Mux23/3
  [c_rr_t] -> Mux23/1
  [th_rr_t] -> Mux23/2
  [th_rm_t] -> Mux28/2
  [c_rm_t] -> Mux28/1
  [t_rm_t] -> Mux28/3
  [t_rf_t] -> Mux27/3
  [c_rf_t] -> Mux27/1
  Mux27/1 -> Mux3/4
  [c_lm_t] -> Mux25/1
  [t_lm_t] -> Mux25/3
  Mux26/1 -> Mux3/3
  [th_lf_t] -> Mux24/2
  [th_lm_t] -> Mux25/2
  [c_lf_t] -> Mux24/1
  [th_rf_t] -> Mux27/2
  Mux24/1 -> Mux3/1
  [t_lr_t] -> Mux26/3
  Mux23/1 -> Mux3/6
  Subtract/1 -> Demux1/1
  Demux1/1 -> Abs/1
  Demux1/2 -> Abs1/1
  Demux1/3 -> Abs2/1
  Demux1/4 -> Abs3/1
  Demux1/5 -> Abs4/1
  Demux1/6 -> Abs5/1
  Demux1/7 -> Abs6/1
  Demux1/8 -> Abs7/1
  Demux1/9 -> Abs8/1
  Demux1/10 -> Abs9/1
  Demux1/11 -> Abs10/1
  Demux1/12 -> Abs11/1
  Demux1/13 -> Abs12/1
  Demux1/14 -> Abs13/1
  Demux1/15 -> Abs14/1
  Demux1/16 -> Abs15/1
  Demux1/17 -> Abs16/1
  Demux1/18 -> Abs17/1
  Constant/1 -> [t_threshold]
  [t_threshold] -> Relational Operator/2
  [t_threshold] -> Relational Operator1/2
  Abs/1 -> Mux29/1
  Abs1/1 -> Mux29/2
  Abs2/1 -> Mux29/3
  Mux29/1 -> Scope6/1, Relational Operator/1
  Abs3/1 -> Mux30/1
  Abs4/1 -> Mux30/2
  Abs5/1 -> Mux30/3
  Mux30/1 -> Scope6/2, Relational Operator1/1
  Mux31/1 -> Scope6/3, Relational Operator2/1
  [t_threshold] -> Relational Operator2/2
  Abs6/1 -> Mux31/1
  Abs7/1 -> Mux31/2
  Abs8/1 -> Mux31/3
  [t_threshold] -> Relational Operator3/2
  Abs9/1 -> Mux32/1
  Abs10/1 -> Mux32/2
  Abs11/1 -> Mux32/3
  Abs12/1 -> Mux33/1
  Abs13/1 -> Mux33/2
  Abs14/1 -> Mux33/3
  Mux34/1 -> Scope6/6, Relational Operator4/1
  [t_threshold] -> Relational Operator4/2
  Abs15/1 -> Mux34/1
  Abs16/1 -> Mux34/2
  Abs17/1 -> Mux34/3
  Mux33/1 -> Scope6/5, Relational Operator5/1
  [t_threshold] -> Relational Operator5/2
  Relational Operator/1 -> Demux2/1
  Demux2/1 -> OR/1
  Demux2/2 -> OR/2
  Demux2/3 -> OR/3
  Demux3/3 -> OR1/3
  Demux3/1 -> OR1/1
  Demux3/2 -> OR1/2
  Relational Operator1/1 -> Demux3/1
  Demux4/3 -> OR2/3
  Demux4/1 -> OR2/1
  Demux4/2 -> OR2/2
  Relational Operator2/1 -> Demux4/1
  Demux5/3 -> OR3/3
  Demux5/1 -> OR3/1
  Demux5/2 -> OR3/2
  Relational Operator3/1 -> Demux5/1
  Demux6/3 -> OR4/3
  Demux6/1 -> OR4/1
  Demux6/2 -> OR4/2
  Relational Operator5/1 -> Demux6/1
  Demux7/3 -> OR5/3
  Demux7/1 -> OR5/1
  Demux7/2 -> OR5/2
  Relational Operator4/1 -> Demux7/1
  OR/1 -> Scope2/1, [cont_lf]
  OR1/1 -> Scope2/2, [cont_lm]
  OR2/1 -> [cont_lr], Scope2/3
  OR3/1 -> [cont_rf], Scope2/4
  OR4/1 -> [cont_rm], Scope2/5
  OR5/1 -> [cont_rr], Scope2/6
  Demux/4 -> Scope/4
  Demux/5 -> Scope/5
  Demux/6 -> Scope/6
  [Force_sens_lf] -> Scope3/1, Mux35/1
  [Force_sens_lm] -> Scope3/2, Mux35/2
  [Force_sens_lr] -> Scope3/3, Mux35/3
  [Force_sens_rf] -> Mux35/4, Scope3/4
  [Force_sens_rm] -> Mux35/5, Scope3/5
  [Force_sens_rr] -> Mux35/6, Scope3/6
  Add1/1 -> To Workspace2/1, Scope4/1  "Fsum"
  From127/1 -> Add1/1
  From128/1 -> Add1/2
  From129/1 -> Add1/3
  From130/1 -> Add1/4
  From131/1 -> Add1/5
  From132/1 -> Add1/6
  Constant1/1 -> MATLAB Function1/6(duty), MATLAB Function/6(duty)
  Mux35/1 -> To Workspace3/1
  Mux32/1 -> Scope6/4, Relational Operator3/1
  [z1] -> MATLAB Function2/1(z)
  MATLAB Function2/1(z_lf) -> [z_lf]
  MATLAB Function2/2(z_lr) -> [z_lr]
  MATLAB Function2/3(z_rm) -> [z_rm]
  Clock2/1 -> MATLAB Function2/5(t)
  [cont_lf] -> Unit Delay/1
  Unit Delay/1 -> MATLAB Function2/2(c_lf)
  [cont_lr] -> Unit Delay1/1
  Unit Delay1/1 -> MATLAB Function2/3(c_lr)
  [cont_rm] -> Unit Delay2/1
  Unit Delay2/1 -> MATLAB Function2/4(c_rm)
  [cont_lm] -> Unit Delay3/1
  Clock3/1 -> MATLAB Function3/5(t)
  [cont_rf] -> Unit Delay4/1
  [cont_rr] -> Unit Delay5/1
  [z2] -> MATLAB Function3/1(z)
  [z_lf] -> Scope8/1
  [z_lm] -> Scope8/2
  [z_lr] -> Scope8/3
  [z_rf] -> Scope8/4
  [z_rm] -> Scope8/5
  [z_rr] -> Scope8/6
  [z_lf] -> To Workspace4/1
  [z_lm] -> To Workspace5/1
  [z_lr] -> To Workspace6/1
  [z_rf] -> To Workspace7/1
  [z_rm] -> To Workspace8/1
  [z_rr] -> To Workspace9/1
  [cont_lf] -> To Workspace10/1
  [cont_lm] -> To Workspace11/1
  [cont_lr] -> To Workspace12/1
  [cont_rf] -> To Workspace13/1
  [cont_rm] -> To Workspace14/1
  [cont_rr] -> To Workspace15/1
  MATLAB Function3/1(z_rf) -> [z_rf]
  MATLAB Function3/2(z_rr) -> [z_rr]
  MATLAB Function3/3(z_lm) -> [z_lm]
  Unit Delay3/1 -> MATLAB Function3/4(c_lm)
  Unit Delay4/1 -> MATLAB Function3/2(c_rf)
  Unit Delay5/1 -> MATLAB Function3/3(c_rr)
  Constant10/1 -> MATLAB Function2/6(par)
  Constant11/1 -> MATLAB Function3/6(par)
  PS-Simulink Converter75/1 -> [Force_sens_rr]
  PS-Simulink Converter76/1 -> [Force_sens_rm]
  PS-Simulink Converter77/1 -> [Force_sens_rf]
  PS-Simulink Converter78/1 -> [Force_sens_lr]
  PS-Simulink Converter79/1 -> [Force_sens_lm]
  PS-Simulink Converter80/1 -> [Force_sens_lf]
  Demux8/1 -> Z/1
  Demux8/2 -> [pitch], Y/1
  Demux8/3 -> X/1
  [pitch] -> Unit Delay6/1
  Sum1/1 -> PID Controller/1
  Constant12/1 -> Sum1/1
  PID Controller/1 -> MATLAB Function4/1(u_theta)
  MATLAB Function4/1(delta_z) -> Demux9/1
  Demux9/1 -> [d_z_lf]
  Demux9/2 -> [d_z_lm]
  Demux9/3 -> [d_z_lr]
  Demux9/4 -> [d_z_rr]
  Demux9/5 -> [d_z_rm]
  Demux9/6 -> [d_z_rf]
  [z_rr] -> Sum2/1
  [z_rm] -> Sum3/1
  Sum3/1 -> Saturation1/1
  [z_rf] -> Sum4/1
  Sum4/1 -> Saturation2/1
  [z_lr] -> Sum5/1
  [z_lm] -> Sum6/1
  [z_lf] -> Sum7/1
  Sum7/1 -> Saturation5/1
  [d_z_rr] -> Sum2/2
  [d_z_rm] -> Sum3/2
  [d_z_rf] -> Sum4/2
  [d_z_lr] -> Sum5/2
  [d_z_lm] -> Sum6/2
  [d_z_lf] -> Sum7/2
  Unit Delay6/1 -> Sum1/2
  Saturation/1 -> Rate Limiter2/1
  Sum2/1 -> Saturation/1
  Saturation2/1 -> Rate Limiter1/1
  Sum5/1 -> Saturation3/1
  Sum6/1 -> Saturation4/1
  Saturation3/1 -> Rate Limiter/1
  Rate Limiter/1 -> Scope9/1, RL/3(z)
  Rate Limiter1/1 -> FR/3(z)
  Rate Limiter2/1 -> RR/3(z)
  Rate Limiter3/1 -> MR/3(z)
  Saturation1/1 -> Rate Limiter3/1
  Saturation4/1 -> Rate Limiter4/1
  Rate Limiter4/1 -> ML/3(z)
  Rate Limiter5/1 -> FL/3(z)
  Saturation5/1 -> Rate Limiter5/1
  connections:
  MP_BODY/LConn1 -- j_phantomx_attachment/RConn1 -- Transform Sensor/RConn1
  MP_BODY/RConn6 -- j_c1_lf/LConn1
  c1_lm/LConn1 -- j_c1_lm/RConn1
  c1_lm/RConn1 -- j_c2_lm/LConn1
  c1_lr/LConn1 -- j_c1_lr/RConn1
  c1_lr/RConn1 -- j_c2_lr/LConn1
  c1_rf/LConn1 -- j_c1_rf/RConn1
  c1_rf/RConn1 -- j_c2_rf/LConn1
  c1_rm/LConn1 -- j_c1_rm/RConn1
  c1_rm/RConn1 -- j_c2_rm/LConn1
  c1_rr/LConn1 -- j_c1_rr/RConn1
  c1_rr/RConn1 -- j_c2_rr/LConn1
  MP_BODY/RConn5 -- j_c1_lm/LConn1
  c2_lf/LConn1 -- j_c2_lf/RConn1
  c2_lf/RConn1 -- j_thigh_lf/LConn1
  c2_lm/LConn1 -- j_c2_lm/RConn1
  c2_lm/RConn1 -- j_thigh_lm/LConn1
  c2_lr/LConn1 -- j_c2_lr/RConn1
  c2_lr/RConn1 -- j_thigh_lr/LConn1
  c2_rf/LConn1 -- j_c2_rf/RConn1
  c2_rf/RConn1 -- j_thigh_rf/LConn1
  c2_rm/LConn1 -- j_c2_rm/RConn1
  c2_rm/RConn1 -- j_thigh_rm/LConn1
  MP_BODY/RConn4 -- j_c1_lr/LConn1
  c2_rr/LConn1 -- j_c2_rr/RConn1
  c2_rr/RConn1 -- j_thigh_rr/LConn1
  j_thigh_lf/RConn1 -- thigh_lf/LConn1
  j_tibia_lf/LConn1 -- thigh_lf/RConn1
  j_thigh_lm/RConn1 -- thigh_lm/LConn1
  j_tibia_lm/LConn1 -- thigh_lm/RConn1
  j_thigh_lr/RConn1 -- thigh_lr/LConn1
  j_tibia_lr/LConn1 -- thigh_lr/RConn1
  j_thigh_rf/RConn1 -- thigh_rf/LConn1
  j_tibia_rf/LConn1 -- thigh_rf/RConn1
  MP_BODY/RConn3 -- j_c1_rf/LConn1
  j_thigh_rm/RConn1 -- thigh_rm/LConn1
  j_tibia_rm/LConn1 -- thigh_rm/RConn1
  j_thigh_rr/RConn1 -- thigh_rr/LConn1
  j_tibia_rr/LConn1 -- thigh_rr/RConn1
  j_tibia_lf/RConn1 -- Rigid Transform6/RConn1 -- tibia_lf/LConn1
  j_tibia_lm/RConn1 -- Rigid Transform5/RConn1 -- tibia_lm/LConn1
  j_tibia_lr/RConn1 -- Rigid Transform4/RConn1 -- tibia_lr/LConn1
  j_tibia_rf/RConn1 -- Rigid Transform1/RConn1 -- tibia_rf/LConn1
  j_tibia_rm/RConn1 -- tibia_rm/LConn1 -- Rigid Transform2/RConn1
  MP_BODY/RConn2 -- j_c1_rm/LConn1
  MechanismConfiguration/RConn1 -- Rigid Transform_Rampa/RConn1 -- Rigid Transform16/RConn1 -- Rigid Transform15/RConn1 -- Rigid Transform14/RConn1 -- Rigid Transform13/RConn1 -- Rigid Transform12/RConn1 -- Rigid Transform11/RConn1 -- Rigid Transform10/RConn1 -- Rigid Transform/RConn1 -- Solver Configuration/RConn1 -- Transform Sensor/LConn1 -- 6-DOF Joint/LConn1 -- World/RConn1
  MP_BODY/RConn1 -- j_c1_rr/LConn1
  base_link/RConn1 -- j_phantomx_attachment/LConn1
  c1_lf/LConn1 -- j_c1_lf/RConn1
  c1_lf/RConn1 -- j_c2_lf/LConn1
  j_c1_rr/RConn2 -- PS-Simulink Converter/LConn1
  Transform Sensor/RConn3 -- PS-Simulink Converter19/LConn1
  PS-Simulink Converter3/LConn1 -- j_thigh_rr/RConn2
  PS-Simulink Converter4/LConn1 -- j_tibia_rr/RConn2
  j_c1_rm/RConn2 -- PS-Simulink Converter7/LConn1
  j_thigh_rm/RConn2 -- PS-Simulink Converter8/LConn1
  PS-Simulink Converter9/LConn1 -- j_tibia_rm/RConn2
  j_c1_rf/RConn2 -- PS-Simulink Converter5/LConn1
  j_thigh_rf/RConn2 -- PS-Simulink Converter20/LConn1
  PS-Simulink Converter6/LConn1 -- j_tibia_rf/RConn2
  j_thigh_lr/RConn2 -- PS-Simulink Converter11/LConn1
  PS-Simulink Converter12/LConn1 -- j_tibia_lr/RConn2
  j_c1_lr/RConn2 -- PS-Simulink Converter10/LConn1
  j_c1_lm/RConn2 -- PS-Simulink Converter13/LConn1
  j_thigh_lm/RConn2 -- PS-Simulink Converter14/LConn1
  j_tibia_lm/RConn2 -- PS-Simulink Converter15/LConn1
  j_c1_lf/RConn2 -- PS-Simulink Converter16/LConn1
  j_thigh_lf/RConn2 -- PS-Simulink Converter17/LConn1
  PS-Simulink Converter18/LConn1 -- j_tibia_lf/RConn2
  Transform Sensor/RConn2 -- PS-Simulink Converter1/LConn1
  Simulink-PS Converter/RConn1 -- j_c1_rr/LConn2
  j_tibia_rr/LConn2 -- Simulink-PS Converter2/RConn1
  Simulink-PS Converter3/RConn1 -- j_c1_rm/LConn2
  j_thigh_rm/LConn2 -- Simulink-PS Converter4/RConn1
  j_tibia_rr/RConn1 -- Rigid Transform3/RConn1 -- tibia_rr/LConn1
  Simulink-PS Converter8/RConn1 -- j_c1_lm/LConn2
  Simulink-PS Converter9/RConn1 -- j_c1_lf/LConn2
  Simulink-PS Converter25/RConn1 -- j_thigh_lf/LConn2
  Simulink-PS Converter23/RConn1 -- j_thigh_lm/LConn2
  Simulink-PS Converter21/RConn1 -- j_thigh_lr/LConn2
  j_tibia_lr/LConn2 -- Simulink-PS Converter20/RConn1
  Simulink-PS Converter22/RConn1 -- j_tibia_lm/LConn2
  Simulink-PS Converter24/RConn1 -- j_tibia_lf/LConn2
  Simulink-PS Converter1/RConn1 -- j_thigh_rr/LConn2
  Simulink-PS Converter18/RConn1 -- j_tibia_rm/LConn2
  Simulink-PS Converter5/RConn1 -- j_c1_rf/LConn2
  Simulink-PS Converter6/RConn1 -- j_c1_lr/LConn2
  Simulink-PS Converter7/RConn1 -- j_thigh_rf/LConn2
  Simulink-PS Converter19/RConn1 -- j_tibia_rf/LConn2
  Rigid Transform/LConn1 -- Solid_Pavimento/RConn1
  Spherical Solid/RConn1 -- Rigid Transform1/LConn1
  Spherical Solid1/RConn1 -- Rigid Transform2/LConn1
  Spherical Solid2/RConn1 -- Rigid Transform3/LConn1
  Spherical Solid3/RConn1 -- Rigid Transform4/LConn1
  Spherical Solid4/RConn1 -- Rigid Transform5/LConn1
  Spherical Solid5/RConn1 -- Rigid Transform6/LConn1
  Connection Label/LConn1 -- Solid_Pavimento/LConn1
  Transform Sensor/RConn4 -- PS-Simulink Converter2/LConn1
  6-DOF Joint/RConn1 -- 6-DOF Joint1/RConn1 -- Brick Solid1/RConn1 -- base_link/LConn1
  PS-Simulink Converter21/LConn1 -- j_c1_rr/RConn3
  PS-Simulink Converter22/LConn1 -- j_thigh_rr/RConn3
  PS-Simulink Converter23/LConn1 -- j_tibia_rr/RConn3
  PS-Simulink Converter24/LConn1 -- j_c1_rr/RConn4
  PS-Simulink Converter25/LConn1 -- j_thigh_rr/RConn4
  PS-Simulink Converter26/LConn1 -- j_tibia_rr/RConn4
  PS-Simulink Converter27/LConn1 -- j_c1_rr/RConn5
  PS-Simulink Converter28/LConn1 -- j_thigh_rr/RConn5
  PS-Simulink Converter29/LConn1 -- j_tibia_rr/RConn5
  PS-Simulink Converter30/LConn1 -- j_c1_rm/RConn3
  PS-Simulink Converter31/LConn1 -- j_c1_rm/RConn4
  PS-Simulink Converter32/LConn1 -- j_c1_rm/RConn5
  PS-Simulink Converter33/LConn1 -- j_c1_rf/RConn3
  PS-Simulink Converter34/LConn1 -- j_c1_rf/RConn4
  PS-Simulink Converter35/LConn1 -- j_c1_rf/RConn5
  PS-Simulink Converter36/LConn1 -- j_c1_lr/RConn3
  PS-Simulink Converter37/LConn1 -- j_c1_lr/RConn4
  PS-Simulink Converter38/LConn1 -- j_c1_lr/RConn5
  j_c1_lm/RConn3 -- PS-Simulink Converter39/LConn1
  PS-Simulink Converter40/LConn1 -- j_c1_lm/RConn4
  PS-Simulink Converter41/LConn1 -- j_c1_lm/RConn5
  PS-Simulink Converter42/LConn1 -- j_c1_lf/RConn3
  PS-Simulink Converter43/LConn1 -- j_c1_lf/RConn4
  PS-Simulink Converter44/LConn1 -- j_c1_lf/RConn5
  PS-Simulink Converter45/LConn1 -- j_thigh_rm/RConn3
  PS-Simulink Converter46/LConn1 -- j_thigh_rm/RConn4
  PS-Simulink Converter47/LConn1 -- j_thigh_rm/RConn5
  j_thigh_rf/RConn3 -- PS-Simulink Converter48/LConn1
  PS-Simulink Converter49/LConn1 -- j_thigh_rf/RConn4
  PS-Simulink Converter50/LConn1 -- j_thigh_rf/RConn5
  PS-Simulink Converter51/LConn1 -- j_thigh_lr/RConn3
  PS-Simulink Converter52/LConn1 -- j_thigh_lr/RConn4
  PS-Simulink Converter53/LConn1 -- j_thigh_lr/RConn5
  PS-Simulink Converter54/LConn1 -- j_thigh_lm/RConn3
  PS-Simulink Converter55/LConn1 -- j_thigh_lm/RConn4
  PS-Simulink Converter56/LConn1 -- j_thigh_lm/RConn5
  PS-Simulink Converter57/LConn1 -- j_thigh_lf/RConn3
  PS-Simulink Converter58/LConn1 -- j_thigh_lf/RConn4
  PS-Simulink Converter59/LConn1 -- j_thigh_lf/RConn5
  PS-Simulink Converter60/LConn1 -- j_tibia_rm/RConn3
  PS-Simulink Converter61/LConn1 -- j_tibia_rm/RConn4
  PS-Simulink Converter62/LConn1 -- j_tibia_rm/RConn5
  PS-Simulink Converter63/LConn1 -- j_tibia_rf/RConn3
  PS-Simulink Converter64/LConn1 -- j_tibia_rf/RConn4
  PS-Simulink Converter65/LConn1 -- j_tibia_rf/RConn5
  PS-Simulink Converter66/LConn1 -- j_tibia_lr/RConn3
  PS-Simulink Converter67/LConn1 -- j_tibia_lr/RConn4
  PS-Simulink Converter68/LConn1 -- j_tibia_lr/RConn5
  PS-Simulink Converter69/LConn1 -- j_tibia_lm/RConn3
  PS-Simulink Converter70/LConn1 -- j_tibia_lm/RConn4
  PS-Simulink Converter71/LConn1 -- j_tibia_lm/RConn5
  PS-Simulink Converter72/LConn1 -- j_tibia_lf/RConn3
  j_tibia_lf/RConn4 -- PS-Simulink Converter73/LConn1
  PS-Simulink Converter74/LConn1 -- j_tibia_lf/RConn5
  Rigid Transform10/LConn1 -- Solid_Ostacolo1/RConn1
  Connection Label16/LConn1 -- Solid_Ostacolo1/LConn1
  Subsystem/RConn1 -- Spherical Solid2/LConn1
  Connection Label1/LConn1 -- Subsystem/LConn1
  Connection Label2/LConn1 -- Subsystem/LConn2
  Connection Label18/LConn1 -- Subsystem/LConn3
  Connection Label17/LConn1 -- Solid_Ostacolo2/LConn1
  Rigid Transform11/LConn1 -- Solid_Ostacolo2/RConn1
  Rigid Transform12/LConn1 -- Solid_Ostacolo3/RConn1
  Connection Label24/LConn1 -- Solid_Ostacolo3/LConn1
  Connection Label25/LConn1 -- Subsystem/LConn4
  Rigid Transform13/LConn1 -- Solid_Ostacolo4/RConn1
  Connection Label31/LConn1 -- Solid_Ostacolo4/LConn1
  Connection Label32/LConn1 -- Subsystem/LConn5
  Connection Label38/LConn1 -- Solid_Ostacolo5/LConn1
  Rigid Transform14/LConn1 -- Solid_Ostacolo5/RConn1
  Connection Label39/LConn1 -- Solid_Ostacolo6/LConn1
  Rigid Transform15/LConn1 -- Solid_Ostacolo6/RConn1
  Connection Label40/LConn1 -- Subsystem/LConn6
  Connection Label41/LConn1 -- Subsystem/LConn7
  Rigid Transform16/LConn1 -- Solid_Ostacolo7/RConn1
  Connection Label12/LConn1 -- Solid_Ostacolo7/LConn1
  Connection Label13/LConn1 -- Subsystem/LConn8
  PS-Simulink Converter75/LConn1 -- Subsystem/RConn2
  Rigid Transform_Rampa/LConn1 -- Solid_Rampa/RConn1
  Connection Label7/LConn1 -- Solid_Rampa/LConn1
  Connection Label3/LConn1 -- Subsystem/LConn9
  Connection Label23/LConn1 -- Subsystem1/LConn4
  Connection Label15/LConn1 -- Subsystem1/LConn3
  Subsystem1/RConn1 -- Spherical Solid1/LConn1
  Connection Label43/LConn1 -- Subsystem1/LConn7
  Connection Label42/LConn1 -- Subsystem1/LConn6
  Connection Label4/LConn1 -- Subsystem1/LConn1
  Connection Label19/LConn1 -- Subsystem1/LConn2
  Connection Label33/LConn1 -- Subsystem1/LConn5
  Connection Label26/LConn1 -- Subsystem1/LConn9
  Connection Label14/LConn1 -- Subsystem1/LConn8
  PS-Simulink Converter76/LConn1 -- Subsystem1/RConn2
  Connection Label10/LConn1 -- Subsystem2/LConn4
  Connection Label8/LConn1 -- Subsystem2/LConn3
  Subsystem2/RConn1 -- Spherical Solid/LConn1
  Connection Label22/LConn1 -- Subsystem2/LConn7
  Connection Label21/LConn1 -- Subsystem2/LConn6
  Connection Label5/LConn1 -- Subsystem2/LConn1
  Connection Label9/LConn1 -- Subsystem2/LConn2
  Connection Label20/LConn1 -- Subsystem2/LConn5
  Connection Label11/LConn1 -- Subsystem2/LConn9
  Connection Label6/LConn1 -- Subsystem2/LConn8
  PS-Simulink Converter77/LConn1 -- Subsystem2/RConn2
  Connection Label34/LConn1 -- Subsystem3/LConn4
  Connection Label29/LConn1 -- Subsystem3/LConn3
  Subsystem3/RConn1 -- Spherical Solid3/LConn1
  Connection Label44/LConn1 -- Subsystem3/LConn7
  Connection Label37/LConn1 -- Subsystem3/LConn6
  Connection Label27/LConn1 -- Subsystem3/LConn1
  Connection Label30/LConn1 -- Subsystem3/LConn2
  Connection Label36/LConn1 -- Subsystem3/LConn5
  Connection Label35/LConn1 -- Subsystem3/LConn9
  Connection Label28/LConn1 -- Subsystem3/LConn8
  PS-Simulink Converter78/LConn1 -- Subsystem3/RConn2
  Connection Label49/LConn1 -- Subsystem4/LConn4
  Connection Label47/LConn1 -- Subsystem4/LConn3
  Subsystem4/RConn1 -- Spherical Solid4/LConn1
  Connection Label53/LConn1 -- Subsystem4/LConn7
  Connection Label52/LConn1 -- Subsystem4/LConn6
  Connection Label45/LConn1 -- Subsystem4/LConn1
  Connection Label48/LConn1 -- Subsystem4/LConn2
  Connection Label51/LConn1 -- Subsystem4/LConn5
  Connection Label50/LConn1 -- Subsystem4/LConn9
  Connection Label46/LConn1 -- Subsystem4/LConn8
  PS-Simulink Converter79/LConn1 -- Subsystem4/RConn2
  Connection Label58/LConn1 -- Subsystem5/LConn4
  Connection Label56/LConn1 -- Subsystem5/LConn3
  Subsystem5/RConn1 -- Spherical Solid5/LConn1
  Connection Label62/LConn1 -- Subsystem5/LConn7
  Connection Label61/LConn1 -- Subsystem5/LConn6
  Connection Label54/LConn1 -- Subsystem5/LConn1
  Connection Label57/LConn1 -- Subsystem5/LConn2
  Connection Label60/LConn1 -- Subsystem5/LConn5
  Connection Label59/LConn1 -- Subsystem5/LConn9
  Connection Label55/LConn1 -- Subsystem5/LConn8
  PS-Simulink Converter80/LConn1 -- Subsystem5/RConn2
  Rigid Transform7/LConn1 -- Brick Solid/RConn1
  Rigid Transform7/RConn1 -- 6-DOF Joint1/LConn1
  Spatial Contact Force/LConn1 -- Brick Solid/LConn1
  Spatial Contact Force/RConn1 -- Brick Solid1/LConn1
